simulink model "myo_sfun_one_myo_imu_emg"  (R2019a)
settings: Solver=ode1  StartTime=0.0  StopTime=inf  FixedStep=0.005  RelTol=1e-3  EnableMultiTasking=on
libraries: neural x1018, myo_lib x2, sldrtlib x1, dspnetwork x1
(part 4 of 12)

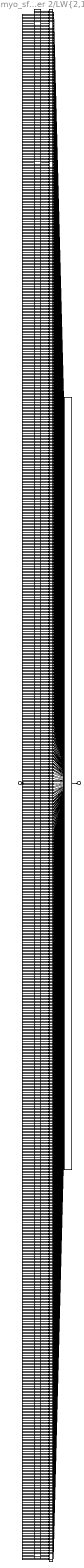
== system myo_sfun_one_myo_imu_emg/Pattern Recognition Neural Network/Layer 2/LW{2,1} ==
  "ad{2,1}" : Inport  PortDimensions=8
      mask Display: e = 0.06;c1 = [120 230 180]/255;c2 = ([120 230 180]+0)/(256+128);c3 = ([120 230 180]+128)/(256+128);patch([0 1 1 0],[0 0 1 1],c1);patch([0 1 1 1-e 1-e 0+e],[0 0 1 1-e 0+e 0+e],c2);patch([0 0 1 1-e 0+e 0+e],[0 1 1 1-e 1-e 0+e],c3);plot([0 1 1 0 0],[0 0 1 1 0]);
  "IW{2,1}(1,:)'" : Constant  Value=[-0.691660917205364711435322533361613750457763671875;-1.7584420611645865673011712715378962457180023193359375;-1.7122805471842796887216309187351725995540618896484375;0.1557580120848369997776927675658953376114368438720703125;-1.4322595499423294018725982823525555431842803955078125;-1.0116917192643277711994187484378926455974578857421875;0.60338568391011870861717625302844680845737457275390625;-1.10261377542594374290274572558701038360595703125]
      mask Display: e = 0.06;c1 = [120 150 230]/255;c2 = ([120 150 230]+0)/383;c3 = ([120 150 230]+128)/383;patch([0 1 1 0],[0 0 1 1],c1);patch([0 1 1 1-e 1-e 0+e],[0 0 1 1-e 0+e 0+e],c2);patch([0 0 1 1-e 0+e 0+e],[0 1 1 1-e 1-e 0+e],c3);plot([0 1 1 0 0],[0 0 1 1 0]);disp('weights');
  "IW{2,1}(10,:)'" : Constant  Value=[0.29748051894865035205128833695198409259319305419921875;-1.4335889907109626850711947554373182356357574462890625;0.162112670099137046175741261322400532662868499755859375;-1.5012829071378430700889339277637191116809844970703125;2.075601849797474418579668054007925093173980712890625;1.3052358877568857042916761201922781765460968017578125;0.2314436321550090436272029137398931197822093963623046875;-0.75565891962408227033876073619467206299304962158203125]
      mask Display: e = 0.06;c1 = [120 150 230]/255;c2 = ([120 150 230]+0)/383;c3 = ([120 150 230]+128)/383;patch([0 1 1 0],[0 0 1 1],c1);patch([0 1 1 1-e 1-e 0+e],[0 0 1 1-e 0+e 0+e],c2);patch([0 0 1 1-e 0+e 0+e],[0 1 1 1-e 1-e 0+e],c3);plot([0 1 1 0 0],[0 0 1 1 0]);disp('weights');
  "IW{2,1}(100,:)'" : Constant  Value=[-0.1965433836533932165924198898210306651890277862548828125;-0.694918414161374897730638622306287288665771484375;0.66443928778979233218393574134097434580326080322265625;0.4810398818895180728105742673506028950214385986328125;-0.77850581457315548572495345069910399615764617919921875;-1.77609819693787951422336846007965505123138427734375;1.4679904515706148071529923981870524585247039794921875;-1.944332630962620545034269525785930454730987548828125]
      mask Display: e = 0.06;c1 = [120 150 230]/255;c2 = ([120 150 230]+0)/383;c3 = ([120 150 230]+128)/383;patch([0 1 1 0],[0 0 1 1],c1);patch([0 1 1 1-e 1-e 0+e],[0 0 1 1-e 0+e 0+e],c2);patch([0 0 1 1-e 0+e 0+e],[0 1 1 1-e 1-e 0+e],c3);plot([0 1 1 0 0],[0 0 1 1 0]);disp('weights');
  "IW{2,1}(1000,:)'" : Constant  Value=[-0.75896391948230645940753902323194779455661773681640625;1.8795374511604172607093232727493159472942352294921875;1.5450884416724310899127203811076469719409942626953125;0.98730253999568906575490245813853107392787933349609375;0.54160434848503913318751301630982197821140289306640625;-1.3842186077384701636816544123576022684574127197265625;-1.0252246817422523417207003149087540805339813232421875;-0.61302757920082961984320490955724380910396575927734375]
      mask Display: e = 0.06;c1 = [120 150 230]/255;c2 = ([120 150 230]+0)/383;c3 = ([120 150 230]+128)/383;patch([0 1 1 0],[0 0 1 1],c1);patch([0 1 1 1-e 1-e 0+e],[0 0 1 1-e 0+e 0+e],c2);patch([0 0 1 1-e 0+e 0+e],[0 1 1 1-e 1-e 0+e],c3);plot([0 1 1 0 0],[0 0 1 1 0]);disp('weights');
  "IW{2,1}(101,:)'" : Constant  Value=[-0.7346292753484846560496634992887265980243682861328125;1.6733957934261258770902713877148926258087158203125;-0.93987189965385997680868968018330633640289306640625;-2.098880370538726225504433386959135532379150390625;0.41553672602720481688010067955474369227886199951171875;0.483898246991799119154364916539634577929973602294921875;-1.4358615101881204711986583788529969751834869384765625;-0.5692919905849540551656673414981923997402191162109375]
      mask Display: e = 0.06;c1 = [120 150 230]/255;c2 = ([120 150 230]+0)/383;c3 = ([120 150 230]+128)/383;patch([0 1 1 0],[0 0 1 1],c1);patch([0 1 1 1-e 1-e 0+e],[0 0 1 1-e 0+e 0+e],c2);patch([0 0 1 1-e 0+e 0+e],[0 1 1 1-e 1-e 0+e],c3);plot([0 1 1 0 0],[0 0 1 1 0]);disp('weights');
  "IW{2,1}(102,:)'" : Constant  Value=[-0.752794916939543146128244188730604946613311767578125;1.166938084302759026655849083908833563327789306640625;2.171459819669392832253151937038637697696685791015625;0.55570154129463655845455605231109075248241424560546875;1.7372623920478691417201844160445034503936767578125;-0.1828342599738930207564635566086508333683013916015625;0.617021132023727769677634569234214723110198974609375;-0.798583301335380912888695092988200485706329345703125]
      mask Display: e = 0.06;c1 = [120 150 230]/255;c2 = ([120 150 230]+0)/383;c3 = ([120 150 230]+128)/383;patch([0 1 1 0],[0 0 1 1],c1);patch([0 1 1 1-e 1-e 0+e],[0 0 1 1-e 0+e 0+e],c2);patch([0 0 1 1-e 0+e 0+e],[0 1 1 1-e 1-e 0+e],c3);plot([0 1 1 0 0],[0 0 1 1 0]);disp('weights');
  "IW{2,1}(103,:)'" : Constant  Value=[-1.1068634406180850593415243565686978399753570556640625;-0.68329593258649257148107380999135784804821014404296875;0.9236877373804779356447625104920007288455963134765625;-0.79483289464276729585634484465117566287517547607421875;-1.36336981772248311273187937331385910511016845703125;-1.6712995505896552916880182237946428358554840087890625;-1.63520965259610573383497467148117721080780029296875;0.7975112275656390803391104782349430024623870849609375]
      mask Display: e = 0.06;c1 = [120 150 230]/255;c2 = ([120 150 230]+0)/383;c3 = ([120 150 230]+128)/383;patch([0 1 1 0],[0 0 1 1],c1);patch([0 1 1 1-e 1-e 0+e],[0 0 1 1-e 0+e 0+e],c2);patch([0 0 1 1-e 0+e 0+e],[0 1 1 1-e 1-e 0+e],c3);plot([0 1 1 0 0],[0 0 1 1 0]);disp('weights');
  "IW{2,1}(104,:)'" : Constant  Value=[-1.2039908850799425632516204132116399705410003662109375;-1.722550343662703209446362961898557841777801513671875;-0.733634489926349164790053691831417381763458251953125;1.482941468037298538007462411769665777683258056640625;0.0976439227042145974078124481820850633084774017333984375;-1.577352115355438844090940619935281574726104736328125;0.4027722868890502017080734731280244886875152587890625;1.4632670973491415100653512126882560551166534423828125]
      mask Display: e = 0.06;c1 = [120 150 230]/255;c2 = ([120 150 230]+0)/383;c3 = ([120 150 230]+128)/383;patch([0 1 1 0],[0 0 1 1],c1);patch([0 1 1 1-e 1-e 0+e],[0 0 1 1-e 0+e 0+e],c2);patch([0 0 1 1-e 0+e 0+e],[0 1 1 1-e 1-e 0+e],c3);plot([0 1 1 0 0],[0 0 1 1 0]);disp('weights');
  "IW{2,1}(105,:)'" : Constant  Value=[-0.82970148356722717153388657607138156890869140625;1.476196773208704460245144218788482248783111572265625;-0.84817603974084032625313511744025163352489471435546875;-1.357590893906548412672918857424519956111907958984375;1.9196514396686323866703105522901751101016998291015625;0.51783204664954884943739443770027719438076019287109375;0.166333228616280137668326233324478380382061004638671875;1.2661311610600314292440771168912760913372039794921875]
      mask Display: e = 0.06;c1 = [120 150 230]/255;c2 = ([120 150 230]+0)/383;c3 = ([120 150 230]+128)/383;patch([0 1 1 0],[0 0 1 1],c1);patch([0 1 1 1-e 1-e 0+e],[0 0 1 1-e 0+e 0+e],c2);patch([0 0 1 1-e 0+e 0+e],[0 1 1 1-e 1-e 0+e],c3);plot([0 1 1 0 0],[0 0 1 1 0]);disp('weights');
  "IW{2,1}(106,:)'" : Constant  Value=[-2.049359601734397795524955654400400817394256591796875;-1.665285450772149733467131227371282875537872314453125;0.87993744188790279370238067713216878473758697509765625;-1.5679190268193672341823230453883297741413116455078125;0.36094306234647299813644849564298056066036224365234375;-0.0369441453771053307519878217135556042194366455078125;0.0216282674490956665358520893960303510539233684539794921875;-0.99199514984426906405445834025158546864986419677734375]
      mask Display: e = 0.06;c1 = [120 150 230]/255;c2 = ([120 150 230]+0)/383;c3 = ([120 150 230]+128)/383;patch([0 1 1 0],[0 0 1 1],c1);patch([0 1 1 1-e 1-e 0+e],[0 0 1 1-e 0+e 0+e],c2);patch([0 0 1 1-e 0+e 0+e],[0 1 1 1-e 1-e 0+e],c3);plot([0 1 1 0 0],[0 0 1 1 0]);disp('weights');
  "IW{2,1}(107,:)'" : Constant  Value=[1.526235863593053299069879358285106718540191650390625;-1.2098465596567213875545121481991373002529144287109375;-0.3327773356104037905112136286334134638309478759765625;1.6991612055741971420985692020622082054615020751953125;-1.4350855371585951036905726141412742435932159423828125;0.09974716737212674377843768525053746998310089111328125;-1.0362891110155614260435186224640347063541412353515625;1.13218572804818240484792113420553505420684814453125]
      mask Display: e = 0.06;c1 = [120 150 230]/255;c2 = ([120 150 230]+0)/383;c3 = ([120 150 230]+128)/383;patch([0 1 1 0],[0 0 1 1],c1);patch([0 1 1 1-e 1-e 0+e],[0 0 1 1-e 0+e 0+e],c2);patch([0 0 1 1-e 0+e 0+e],[0 1 1 1-e 1-e 0+e],c3);plot([0 1 1 0 0],[0 0 1 1 0]);disp('weights');
  "IW{2,1}(108,:)'" : Constant  Value=[-0.8124994162632557248571174568496644496917724609375;-1.5665539983796381573455391844618134200572967529296875;-0.187224386217166360868446872700587846338748931884765625;1.0861775880444961561721584075712598860263824462890625;1.351917275444545651907901628874242305755615234375;-0.83378037725782350175762758226483128964900970458984375;-1.385421527250217277327237752615474164485931396484375;1.5546422525807359615868108448921702802181243896484375]
      mask Display: e = 0.06;c1 = [120 150 230]/255;c2 = ([120 150 230]+0)/383;c3 = ([120 150 230]+128)/383;patch([0 1 1 0],[0 0 1 1],c1);patch([0 1 1 1-e 1-e 0+e],[0 0 1 1-e 0+e 0+e],c2);patch([0 0 1 1-e 0+e 0+e],[0 1 1 1-e 1-e 0+e],c3);plot([0 1 1 0 0],[0 0 1 1 0]);disp('weights');
  "IW{2,1}(109,:)'" : Constant  Value=[0.19012578102685784298131466130143962800502777099609375;1.44821196542192875966748033533804118633270263671875;-0.669229510490122248000943727674894034862518310546875;1.3059840050621274176734232241869904100894927978515625;-0.8163339678271857025038116262294352054595947265625;-1.4775762628706907708675544199650175869464874267578125;0.87987224253331641765640824814909137785434722900390625;1.6788826743721418921495569520629942417144775390625]
      mask Display: e = 0.06;c1 = [120 150 230]/255;c2 = ([120 150 230]+0)/383;c3 = ([120 150 230]+128)/383;patch([0 1 1 0],[0 0 1 1],c1);patch([0 1 1 1-e 1-e 0+e],[0 0 1 1-e 0+e 0+e],c2);patch([0 0 1 1-e 0+e 0+e],[0 1 1 1-e 1-e 0+e],c3);plot([0 1 1 0 0],[0 0 1 1 0]);disp('weights');
  "IW{2,1}(11,:)'" : Constant  Value=[2.091364144074137954021352925337851047515869140625;1.19190169735374329462729292572475969791412353515625;0.438539695265063256268689428907237015664577484130859375;1.427779135746976901799598635989241302013397216796875;-1.1734334596731803568303575957543216645717620849609375;-0.75612406354167938093979728364502079784870147705078125;-0.85559840138312071022852478563436307013034820556640625;0.6340354257080207389662973582744598388671875]
      mask Display: e = 0.06;c1 = [120 150 230]/255;c2 = ([120 150 230]+0)/383;c3 = ([120 150 230]+128)/383;patch([0 1 1 0],[0 0 1 1],c1);patch([0 1 1 1-e 1-e 0+e],[0 0 1 1-e 0+e 0+e],c2);patch([0 0 1 1-e 0+e 0+e],[0 1 1 1-e 1-e 0+e],c3);plot([0 1 1 0 0],[0 0 1 1 0]);disp('weights');
  "IW{2,1}(110,:)'" : Constant  Value=[1.12310065411607507002145212027244269847869873046875;0.65381754150688775606425906516960822045803070068359375;0.483190932248633464585196861662552691996097564697265625;1.5216055898993252615269966554478742182254791259765625;-1.618210254067223186069668372510932385921478271484375;-0.8486399726322251257926154721644707024097442626953125;0.424500550557350420088909004334709607064723968505859375;1.760175767722318429520100835361517965793609619140625]
      mask Display: e = 0.06;c1 = [120 150 230]/255;c2 = ([120 150 230]+0)/383;c3 = ([120 150 230]+128)/383;patch([0 1 1 0],[0 0 1 1],c1);patch([0 1 1 1-e 1-e 0+e],[0 0 1 1-e 0+e 0+e],c2);patch([0 0 1 1-e 0+e 0+e],[0 1 1 1-e 1-e 0+e],c3);plot([0 1 1 0 0],[0 0 1 1 0]);disp('weights');
  "IW{2,1}(111,:)'" : Constant  Value=[-1.45835723777261261346893661539070308208465576171875;0.460958016356734834317876448039896786212921142578125;0.82960262943399343260608702621539123356342315673828125;1.764946563170818993881994174444116652011871337890625;1.867300072530361010336719118640758097171783447265625;0.4866543505420615201018108564312569797039031982421875;0.47638255663761619462803764690761454403400421142578125;0.967658595669160792596130704623647034168243408203125]
      mask Display: e = 0.06;c1 = [120 150 230]/255;c2 = ([120 150 230]+0)/383;c3 = ([120 150 230]+128)/383;patch([0 1 1 0],[0 0 1 1],c1);patch([0 1 1 1-e 1-e 0+e],[0 0 1 1-e 0+e 0+e],c2);patch([0 0 1 1-e 0+e 0+e],[0 1 1 1-e 1-e 0+e],c3);plot([0 1 1 0 0],[0 0 1 1 0]);disp('weights');
  "IW{2,1}(112,:)'" : Constant  Value=[0.90630292675991774853372362485970370471477508544921875;-0.7483178408217094901289101471775211393833160400390625;-1.4719554269169139448791838731267489492893218994140625;-1.3185905102969688318381713543203659355640411376953125;1.11248064428886461740830782218836247920989990234375;-1.902432566793907486868420164682902395725250244140625;0.80968802704409836845655945580801926553249359130859375;0.471445922634182945643033235683105885982513427734375]
      mask Display: e = 0.06;c1 = [120 150 230]/255;c2 = ([120 150 230]+0)/383;c3 = ([120 150 230]+128)/383;patch([0 1 1 0],[0 0 1 1],c1);patch([0 1 1 1-e 1-e 0+e],[0 0 1 1-e 0+e 0+e],c2);patch([0 0 1 1-e 0+e 0+e],[0 1 1 1-e 1-e 0+e],c3);plot([0 1 1 0 0],[0 0 1 1 0]);disp('weights');
  "IW{2,1}(113,:)'" : Constant  Value=[-2.1700138842824419072030650568194687366485595703125;-1.2265632677169240327685884039965458214282989501953125;0.31278242318674431832192794900038279592990875244140625;-1.17937237170043918155215578735806047916412353515625;0.495421493364235576706278152414597570896148681640625;1.579508580603393941288459245697595179080963134765625;-0.435311629212086825813088353243074379861354827880859375;0.6223682610868095377298914172570221126079559326171875]
      mask Display: e = 0.06;c1 = [120 150 230]/255;c2 = ([120 150 230]+0)/383;c3 = ([120 150 230]+128)/383;patch([0 1 1 0],[0 0 1 1],c1);patch([0 1 1 1-e 1-e 0+e],[0 0 1 1-e 0+e 0+e],c2);patch([0 0 1 1-e 0+e 0+e],[0 1 1 1-e 1-e 0+e],c3);plot([0 1 1 0 0],[0 0 1 1 0]);disp('weights');
  "IW{2,1}(114,:)'" : Constant  Value=[-0.95960652512177302408957757506868802011013031005859375;-1.171099316170392423686053007259033620357513427734375;1.2005938613692059835358350028400309383869171142578125;-1.0271322442187591494899834287934936583042144775390625;0.275734884241691513562244608692708425223827362060546875;-2.273917403532263126209045367431826889514923095703125;0.60594431945872850864276415450149215757846832275390625;0.788812091891621047778926367755047976970672607421875]
      mask Display: e = 0.06;c1 = [120 150 230]/255;c2 = ([120 150 230]+0)/383;c3 = ([120 150 230]+128)/383;patch([0 1 1 0],[0 0 1 1],c1);patch([0 1 1 1-e 1-e 0+e],[0 0 1 1-e 0+e 0+e],c2);patch([0 0 1 1-e 0+e 0+e],[0 1 1 1-e 1-e 0+e],c3);plot([0 1 1 0 0],[0 0 1 1 0]);disp('weights');
  "IW{2,1}(115,:)'" : Constant  Value=[1.259842960302490322277435552678070962429046630859375;1.7763440982486831121178738612798042595386505126953125;1.7368956039236851385254567503579892218112945556640625;0.489479457804314399549383551857317797839641571044921875;-0.69836997846389603505912191394600085914134979248046875;-0.69450858609234611407146076089702546596527099609375;-1.584018966753015345005906056030653417110443115234375;-0.143556776088628101906152778610703535377979278564453125]
      mask Display: e = 0.06;c1 = [120 150 230]/255;c2 = ([120 150 230]+0)/383;c3 = ([120 150 230]+128)/383;patch([0 1 1 0],[0 0 1 1],c1);patch([0 1 1 1-e 1-e 0+e],[0 0 1 1-e 0+e 0+e],c2);patch([0 0 1 1-e 0+e 0+e],[0 1 1 1-e 1-e 0+e],c3);plot([0 1 1 0 0],[0 0 1 1 0]);disp('weights');
  "IW{2,1}(116,:)'" : Constant  Value=[1.1305890114884669106487535827909596264362335205078125;-0.2309211402775909471873916345430188812315464019775390625;1.4467085200288185564687637452152557671070098876953125;1.683074804270280555584804460522718727588653564453125;-1.10822346900712087602869360125623643398284912109375;1.3197346249344026336558499679085798561573028564453125;0.19679073836889859894228038683650083839893341064453125;-1.310618823194344084726026267162524163722991943359375]
      mask Display: e = 0.06;c1 = [120 150 230]/255;c2 = ([120 150 230]+0)/383;c3 = ([120 150 230]+128)/383;patch([0 1 1 0],[0 0 1 1],c1);patch([0 1 1 1-e 1-e 0+e],[0 0 1 1-e 0+e 0+e],c2);patch([0 0 1 1-e 0+e 0+e],[0 1 1 1-e 1-e 0+e],c3);plot([0 1 1 0 0],[0 0 1 1 0]);disp('weights');
  "IW{2,1}(117,:)'" : Constant  Value=[-1.2965092749014439643673313184990547597408294677734375;-0.40909004021247497018265448787133209407329559326171875;0.232380826221318004254356992532848380506038665771484375;-1.4938038430410289780780885848798789083957672119140625;-1.4111858515245507827984283721889369189739227294921875;-1.3798668297073295452292995832976885139942169189453125;-0.5736035650808333219430323879350908100605010986328125;1.545401209062778224989642694708891212940216064453125]
      mask Display: e = 0.06;c1 = [120 150 230]/255;c2 = ([120 150 230]+0)/383;c3 = ([120 150 230]+128)/383;patch([0 1 1 0],[0 0 1 1],c1);patch([0 1 1 1-e 1-e 0+e],[0 0 1 1-e 0+e 0+e],c2);patch([0 0 1 1-e 0+e 0+e],[0 1 1 1-e 1-e 0+e],c3);plot([0 1 1 0 0],[0 0 1 1 0]);disp('weights');
  "IW{2,1}(118,:)'" : Constant  Value=[-0.431220772164270016446607769466936588287353515625;1.4980663049915936557709983389941044151782989501953125;-0.032124284553384778451157188783327001146972179412841796875;-0.99178065612847543519592363736592233180999755859375;-0.90983063362129545925682805318501777946949005126953125;-0.94491687952873892886174189698067493736743927001953125;0.2190608048581546840605227544074296019971370697021484375;2.4177856342907144693299414939247071743011474609375]
      mask Display: e = 0.06;c1 = [120 150 230]/255;c2 = ([120 150 230]+0)/383;c3 = ([120 150 230]+128)/383;patch([0 1 1 0],[0 0 1 1],c1);patch([0 1 1 1-e 1-e 0+e],[0 0 1 1-e 0+e 0+e],c2);patch([0 0 1 1-e 0+e 0+e],[0 1 1 1-e 1-e 0+e],c3);plot([0 1 1 0 0],[0 0 1 1 0]);disp('weights');
  "IW{2,1}(119,:)'" : Constant  Value=[2.032289941457469328867091462598182260990142822265625;1.2300087485055588576443597048637457191944122314453125;1.1312373102641062327933241249411366879940032958984375;-1.366286246477192545256684752530418336391448974609375;-0.392858662961971472071809330373071134090423583984375;1.3600255209509413134583155624568462371826171875;-0.4417275309143331440964175271801650524139404296875;-0.64492461423233715667180376840406097471714019775390625]
      mask Display: e = 0.06;c1 = [120 150 230]/255;c2 = ([120 150 230]+0)/383;c3 = ([120 150 230]+128)/383;patch([0 1 1 0],[0 0 1 1],c1);patch([0 1 1 1-e 1-e 0+e],[0 0 1 1-e 0+e 0+e],c2);patch([0 0 1 1-e 0+e 0+e],[0 1 1 1-e 1-e 0+e],c3);plot([0 1 1 0 0],[0 0 1 1 0]);disp('weights');
  "IW{2,1}(12,:)'" : Constant  Value=[0.91486769312648663632359102848567999899387359619140625;0.56602701691960033425488063585362397134304046630859375;-1.25438509677780274387259851209819316864013671875;-0.63813074054059371054137272949446924030780792236328125;-1.363451099083925033284003802691586315631866455078125;-0.0252649558450613286042507610318352817557752132415771484375;-2.32042882861984889331097292597405612468719482421875;0.80044852883130257481525404728017747402191162109375]
      mask Display: e = 0.06;c1 = [120 150 230]/255;c2 = ([120 150 230]+0)/383;c3 = ([120 150 230]+128)/383;patch([0 1 1 0],[0 0 1 1],c1);patch([0 1 1 1-e 1-e 0+e],[0 0 1 1-e 0+e 0+e],c2);patch([0 0 1 1-e 0+e 0+e],[0 1 1 1-e 1-e 0+e],c3);plot([0 1 1 0 0],[0 0 1 1 0]);disp('weights');
  "IW{2,1}(120,:)'" : Constant  Value=[0.42250540399770775135124267762876115739345550537109375;1.7440741240887638330292475075111724436283111572265625;1.45134468863258181414721548208035528659820556640625;-0.94540168936672552835176475127809680998325347900390625;1.349986197984198721400161957717500627040863037109375;-0.65996498605669351444902304137940518558025360107421875;-1.73587667519844845998022719868458807468414306640625;0.59414197129898915772372447463567368686199188232421875]
      mask Display: e = 0.06;c1 = [120 150 230]/255;c2 = ([120 150 230]+0)/383;c3 = ([120 150 230]+128)/383;patch([0 1 1 0],[0 0 1 1],c1);patch([0 1 1 1-e 1-e 0+e],[0 0 1 1-e 0+e 0+e],c2);patch([0 0 1 1-e 0+e 0+e],[0 1 1 1-e 1-e 0+e],c3);plot([0 1 1 0 0],[0 0 1 1 0]);disp('weights');
  "IW{2,1}(121,:)'" : Constant  Value=[0.2953824440974088805234032406588084995746612548828125;0.19947891835721265341163643824984319508075714111328125;-1.7008412375581887232556255185045301914215087890625;-0.70194035735294824096541788094327785074710845947265625;2.00078921034554024771523472736589610576629638671875;-0.171731474879736278893460621475242078304290771484375;0.57037505385167686089431526852422393858432769775390625;1.6685824846776340368847968420595861971378326416015625]
      mask Display: e = 0.06;c1 = [120 150 230]/255;c2 = ([120 150 230]+0)/383;c3 = ([120 150 230]+128)/383;patch([0 1 1 0],[0 0 1 1],c1);patch([0 1 1 1-e 1-e 0+e],[0 0 1 1-e 0+e 0+e],c2);patch([0 0 1 1-e 0+e 0+e],[0 1 1 1-e 1-e 0+e],c3);plot([0 1 1 0 0],[0 0 1 1 0]);disp('weights');
  "IW{2,1}(122,:)'" : Constant  Value=[2.389346377458451797792804427444934844970703125;1.8579702943205924636771442237659357488155364990234375;-1.24041157938239177127570656011812388896942138671875;-0.312204907514915308563985263390350155532360076904296875;0.47345305603977294595097191631793975830078125;0.08085799640160480639128337543297675438225269317626953125;0.425169260567675622031202919970382936298847198486328125;-0.58418175654939208385485471808351576328277587890625]
      mask Display: e = 0.06;c1 = [120 150 230]/255;c2 = ([120 150 230]+0)/383;c3 = ([120 150 230]+128)/383;patch([0 1 1 0],[0 0 1 1],c1);patch([0 1 1 1-e 1-e 0+e],[0 0 1 1-e 0+e 0+e],c2);patch([0 0 1 1-e 0+e 0+e],[0 1 1 1-e 1-e 0+e],c3);plot([0 1 1 0 0],[0 0 1 1 0]);disp('weights');
  "IW{2,1}(123,:)'" : Constant  Value=[0.87447765532420562717419443288235925137996673583984375;-1.404484008896221158835260212072171270847320556640625;0.066383199277035453977902079714112915098667144775390625;-2.14177965994965813223416262189857661724090576171875;-0.35409024524090426666589337401092052459716796875;-0.8321991451194150624104395319591276347637176513671875;-0.1303406369226948469108862127541215158998966217041015625;-1.6968377321111436373257674858905375003814697265625]
      mask Display: e = 0.06;c1 = [120 150 230]/255;c2 = ([120 150 230]+0)/383;c3 = ([120 150 230]+128)/383;patch([0 1 1 0],[0 0 1 1],c1);patch([0 1 1 1-e 1-e 0+e],[0 0 1 1-e 0+e 0+e],c2);patch([0 0 1 1-e 0+e 0+e],[0 1 1 1-e 1-e 0+e],c3);plot([0 1 1 0 0],[0 0 1 1 0]);disp('weights');
  "IW{2,1}(124,:)'" : Constant  Value=[-1.20468773335336098995185238891281187534332275390625;-0.86840097966744733692934232749394141137599945068359375;0.5244983963447131802837475333944894373416900634765625;-1.4107774861939119670495301761548034846782684326171875;1.4946368323390231136471584250102750957012176513671875;-1.358016823143335383150542838848195970058441162109375;-0.63820615731996588326779829003498889505863189697265625;-1.41402043973897217910007384489290416240692138671875]
      mask Display: e = 0.06;c1 = [120 150 230]/255;c2 = ([120 150 230]+0)/383;c3 = ([120 150 230]+128)/383;patch([0 1 1 0],[0 0 1 1],c1);patch([0 1 1 1-e 1-e 0+e],[0 0 1 1-e 0+e 0+e],c2);patch([0 0 1 1-e 0+e 0+e],[0 1 1 1-e 1-e 0+e],c3);plot([0 1 1 0 0],[0 0 1 1 0]);disp('weights');
  "IW{2,1}(125,:)'" : Constant  Value=[-0.506779246737117272658679212327115237712860107421875;0.08469404380268320819968863588655949570238590240478515625;0.96661146073616155405261451960541307926177978515625;2.21984576565986291285526021965779364109039306640625;-0.325247928172124389778474551349063403904438018798828125;-2.141187307560778574355708769871853291988372802734375;0.14891670820092250959731927650864236056804656982421875;0.63327011999696491972855483254534192383289337158203125]
      mask Display: e = 0.06;c1 = [120 150 230]/255;c2 = ([120 150 230]+0)/383;c3 = ([120 150 230]+128)/383;patch([0 1 1 0],[0 0 1 1],c1);patch([0 1 1 1-e 1-e 0+e],[0 0 1 1-e 0+e 0+e],c2);patch([0 0 1 1-e 0+e 0+e],[0 1 1 1-e 1-e 0+e],c3);plot([0 1 1 0 0],[0 0 1 1 0]);disp('weights');
  "IW{2,1}(126,:)'" : Constant  Value=[1.954875514761962307375142700038850307464599609375;0.7484979057490068754532330785878002643585205078125;0.1966880304213210750585716368732391856610774993896484375;-0.23710090993159138594847945569199509918689727783203125;1.134606059769200481213147213566116988658905029296875;2.2163351976999177139759922283701598644256591796875;0.361245693778591447919978918434935621917247772216796875;0.29868377131698398141423922425019554793834686279296875]
      mask Display: e = 0.06;c1 = [120 150 230]/255;c2 = ([120 150 230]+0)/383;c3 = ([120 150 230]+128)/383;patch([0 1 1 0],[0 0 1 1],c1);patch([0 1 1 1-e 1-e 0+e],[0 0 1 1-e 0+e 0+e],c2);patch([0 0 1 1-e 0+e 0+e],[0 1 1 1-e 1-e 0+e],c3);plot([0 1 1 0 0],[0 0 1 1 0]);disp('weights');
  "IW{2,1}(127,:)'" : Constant  Value=[0.7694262528917914512049947006744332611560821533203125;0.858673114136447868105506131541915237903594970703125;-1.9591912322259281697967026047990657389163970947265625;0.7765373081231425889114916571998037397861480712890625;-2.12514482442326624322959105484187602996826171875;-0.51247220026288908822920120655908249318599700927734375;0.66660374982875791882719340719631873071193695068359375;0.2215181162421060445666398663888685405254364013671875]
      mask Display: e = 0.06;c1 = [120 150 230]/255;c2 = ([120 150 230]+0)/383;c3 = ([120 150 230]+128)/383;patch([0 1 1 0],[0 0 1 1],c1);patch([0 1 1 1-e 1-e 0+e],[0 0 1 1-e 0+e 0+e],c2);patch([0 0 1 1-e 0+e 0+e],[0 1 1 1-e 1-e 0+e],c3);plot([0 1 1 0 0],[0 0 1 1 0]);disp('weights');
  "IW{2,1}(128,:)'" : Constant  Value=[-0.4645036239519015897059261988033540546894073486328125;0.0578363955944476149095834216495859436690807342529296875;0.79269376078468878343841197420260868966579437255859375;-0.8815416918189125095040026280912570655345916748046875;0.1192744047821424902000586598660447634756565093994140625;2.060366205871878353406145834014751017093658447265625;-1.99426682885684503077072804444469511508941650390625;-1.1547872117878557052250698689022101461887359619140625]
      mask Display: e = 0.06;c1 = [120 150 230]/255;c2 = ([120 150 230]+0)/383;c3 = ([120 150 230]+128)/383;patch([0 1 1 0],[0 0 1 1],c1);patch([0 1 1 1-e 1-e 0+e],[0 0 1 1-e 0+e 0+e],c2);patch([0 0 1 1-e 0+e 0+e],[0 1 1 1-e 1-e 0+e],c3);plot([0 1 1 0 0],[0 0 1 1 0]);disp('weights');
  "IW{2,1}(129,:)'" : Constant  Value=[-1.7954776257203086675673375793849118053913116455078125;-0.77067172361155000803734083092422224581241607666015625;-1.5025825472358846912612762025673873722553253173828125;-1.474556982392986714813787330058403313159942626953125;0.12129332666747798252782075678624096326529979705810546875;-0.462321049146925344697223181356093846261501312255859375;1.33241983510785733102466110722161829471588134765625;-0.472279832509858110700662336967070586979389190673828125]
      mask Display: e = 0.06;c1 = [120 150 230]/255;c2 = ([120 150 230]+0)/383;c3 = ([120 150 230]+128)/383;patch([0 1 1 0],[0 0 1 1],c1);patch([0 1 1 1-e 1-e 0+e],[0 0 1 1-e 0+e 0+e],c2);patch([0 0 1 1-e 0+e 0+e],[0 1 1 1-e 1-e 0+e],c3);plot([0 1 1 0 0],[0 0 1 1 0]);disp('weights');
  "IW{2,1}(13,:)'" : Constant  Value=[1.4722183686413501391143654473125934600830078125;-1.4533406460287687789190158582641743123531341552734375;-1.6756603659175632881073170210584066808223724365234375;0.1239486161395557950459789253727649338543415069580078125;1.065594255147046975906732768635265529155731201171875;-0.455146428364095967378233353883842937648296356201171875;0.2143238030204172861470368616210180334746837615966796875;-1.5942987059197886168249169713817536830902099609375]
      mask Display: e = 0.06;c1 = [120 150 230]/255;c2 = ([120 150 230]+0)/383;c3 = ([120 150 230]+128)/383;patch([0 1 1 0],[0 0 1 1],c1);patch([0 1 1 1-e 1-e 0+e],[0 0 1 1-e 0+e 0+e],c2);patch([0 0 1 1-e 0+e 0+e],[0 1 1 1-e 1-e 0+e],c3);plot([0 1 1 0 0],[0 0 1 1 0]);disp('weights');
  "IW{2,1}(130,:)'" : Constant  Value=[-0.55363441841454597014404725996428169310092926025390625;0.95680857713087352767189486257848329842090606689453125;-1.255947108543568280225599664845503866672515869140625;2.021771324134128189342618497903458774089813232421875;-0.061796225740531542103273210386760183610022068023681640625;2.0317171954915966836097140912897884845733642578125;0.020301648902267176166613893428802839480340480804443359375;0.07304264326480751357006937496407772414386272430419921875]
      mask Display: e = 0.06;c1 = [120 150 230]/255;c2 = ([120 150 230]+0)/383;c3 = ([120 150 230]+128)/383;patch([0 1 1 0],[0 0 1 1],c1);patch([0 1 1 1-e 1-e 0+e],[0 0 1 1-e 0+e 0+e],c2);patch([0 0 1 1-e 0+e 0+e],[0 1 1 1-e 1-e 0+e],c3);plot([0 1 1 0 0],[0 0 1 1 0]);disp('weights');
  "IW{2,1}(131,:)'" : Constant  Value=[-2.180474603917020193222242596675641834735870361328125;0.72645735914720344084116732119582593441009521484375;1.018870908321010571029319180524908006191253662109375;1.383323172901160358350125534343533217906951904296875;0.4625022964292087035431677577435038983821868896484375;0.64331250774203974085452273357077501714229583740234375;1.0715339161900170328323156354599632322788238525390625;-1.0219064363191299182886950802640058100223541259765625]
      mask Display: e = 0.06;c1 = [120 150 230]/255;c2 = ([120 150 230]+0)/383;c3 = ([120 150 230]+128)/383;patch([0 1 1 0],[0 0 1 1],c1);patch([0 1 1 1-e 1-e 0+e],[0 0 1 1-e 0+e 0+e],c2);patch([0 0 1 1-e 0+e 0+e],[0 1 1 1-e 1-e 0+e],c3);plot([0 1 1 0 0],[0 0 1 1 0]);disp('weights');
  "IW{2,1}(132,:)'" : Constant  Value=[0.75489337030717684751124352260376326739788055419921875;-0.782732462432700781818084578844718635082244873046875;0.5931203619410660987654182463302277028560638427734375;0.9184312361182238593215743094333447515964508056640625;-0.42386247367815510500577147467993199825286865234375;1.56965304535986671652381119201891124248504638671875;1.6982589389750326613892639215919189155101776123046875;1.750190304231196147810578622738830745220184326171875]
      mask Display: e = 0.06;c1 = [120 150 230]/255;c2 = ([120 150 230]+0)/383;c3 = ([120 150 230]+128)/383;patch([0 1 1 0],[0 0 1 1],c1);patch([0 1 1 1-e 1-e 0+e],[0 0 1 1-e 0+e 0+e],c2);patch([0 0 1 1-e 0+e 0+e],[0 1 1 1-e 1-e 0+e],c3);plot([0 1 1 0 0],[0 0 1 1 0]);disp('weights');
  "IW{2,1}(133,:)'" : Constant  Value=[0.7123465712444403408198922988958656787872314453125;2.361424615797688364438045027782209217548370361328125;1.903559317488005664387173965224064886569976806640625;-0.11361441222337249901119804462723550386726856231689453125;0.68170139583434796737293481783126480877399444580078125;0.1784087551198940968522066441437345929443836212158203125;-0.468471511711015142775949016140657477080821990966796875;-0.807410088487492405562306885258294641971588134765625]
      mask Display: e = 0.06;c1 = [120 150 230]/255;c2 = ([120 150 230]+0)/383;c3 = ([120 150 230]+128)/383;patch([0 1 1 0],[0 0 1 1],c1);patch([0 1 1 1-e 1-e 0+e],[0 0 1 1-e 0+e 0+e],c2);patch([0 0 1 1-e 0+e 0+e],[0 1 1 1-e 1-e 0+e],c3);plot([0 1 1 0 0],[0 0 1 1 0]);disp('weights');
  "IW{2,1}(134,:)'" : Constant  Value=[-0.328643765864757797512396564343362115323543548583984375;-1.276933252111870586986697162501513957977294921875;1.097953859945065335779190718312747776508331298828125;-1.153794867206221486100048423395492136478424072265625;-1.5442594975204340101981870247982442378997802734375;1.673469912381605251283644975046627223491668701171875;-1.159139076499020593047362126526422798633575439453125;0.1317811894474552880662798770572408102452754974365234375]
      mask Display: e = 0.06;c1 = [120 150 230]/255;c2 = ([120 150 230]+0)/383;c3 = ([120 150 230]+128)/383;patch([0 1 1 0],[0 0 1 1],c1);patch([0 1 1 1-e 1-e 0+e],[0 0 1 1-e 0+e 0+e],c2);patch([0 0 1 1-e 0+e 0+e],[0 1 1 1-e 1-e 0+e],c3);plot([0 1 1 0 0],[0 0 1 1 0]);disp('weights');
  "IW{2,1}(135,:)'" : Constant  Value=[1.4253380172535343728412726704846136271953582763671875;-0.52469999443522008508722365149878896772861480712890625;1.645781957646773374648319077095948159694671630859375;-0.5149944992681885214125259153661318123340606689453125;0.30444887016464150519823306240141391754150390625;-1.5217037329414615509648456281865946948528289794921875;-1.53829529199834968977711469051428139209747314453125;-0.96248226085746335645154658777755685150623321533203125]
      mask Display: e = 0.06;c1 = [120 150 230]/255;c2 = ([120 150 230]+0)/383;c3 = ([120 150 230]+128)/383;patch([0 1 1 0],[0 0 1 1],c1);patch([0 1 1 1-e 1-e 0+e],[0 0 1 1-e 0+e 0+e],c2);patch([0 0 1 1-e 0+e 0+e],[0 1 1 1-e 1-e 0+e],c3);plot([0 1 1 0 0],[0 0 1 1 0]);disp('weights');
  "IW{2,1}(136,:)'" : Constant  Value=[1.8340364443172740838150502895587123930454254150390625;-0.495139273869659890525696255281218327581882476806640625;-1.2288020217730137861877892646589316427707672119140625;1.5993785216609410770871591012110002338886260986328125;-1.2526876259677326430619359598495066165924072265625;0.1816725225549948863346116922912187874317169189453125;-1.287919742756589602805661343154497444629669189453125;-0.12495088404816152849452493001081165857613086700439453125]
      mask Display: e = 0.06;c1 = [120 150 230]/255;c2 = ([120 150 230]+0)/383;c3 = ([120 150 230]+128)/383;patch([0 1 1 0],[0 0 1 1],c1);patch([0 1 1 1-e 1-e 0+e],[0 0 1 1-e 0+e 0+e],c2);patch([0 0 1 1-e 0+e 0+e],[0 1 1 1-e 1-e 0+e],c3);plot([0 1 1 0 0],[0 0 1 1 0]);disp('weights');
  "IW{2,1}(137,:)'" : Constant  Value=[1.2144320976277389600994638385600410401821136474609375;0.53993669110952635659117504474124871194362640380859375;1.7980873460489430470943261752836406230926513671875;-0.1752594036105314945217514832620508968830108642578125;-1.347683724784759728976268888800404965877532958984375;-1.52405694967661187178009640774689614772796630859375;-1.3216497833904288228268342209048569202423095703125;0.2169042246059575962391363646020181477069854736328125]
      mask Display: e = 0.06;c1 = [120 150 230]/255;c2 = ([120 150 230]+0)/383;c3 = ([120 150 230]+128)/383;patch([0 1 1 0],[0 0 1 1],c1);patch([0 1 1 1-e 1-e 0+e],[0 0 1 1-e 0+e 0+e],c2);patch([0 0 1 1-e 0+e 0+e],[0 1 1 1-e 1-e 0+e],c3);plot([0 1 1 0 0],[0 0 1 1 0]);disp('weights');
  "IW{2,1}(138,:)'" : Constant  Value=[1.93517715523273015065797153511084616184234619140625;1.3891910418285957629080940023413859307765960693359375;0.18419004947108608138961471922812052071094512939453125;0.299581378640679074631947287343791685998439788818359375;-1.552318465180493323174459874280728399753570556640625;-1.512560493036712472303406684659421443939208984375;0.59024612509746832156309892525314353406429290771484375;0.399379929496509744613064185614348389208316802978515625]
      mask Display: e = 0.06;c1 = [120 150 230]/255;c2 = ([120 150 230]+0)/383;c3 = ([120 150 230]+128)/383;patch([0 1 1 0],[0 0 1 1],c1);patch([0 1 1 1-e 1-e 0+e],[0 0 1 1-e 0+e 0+e],c2);patch([0 0 1 1-e 0+e 0+e],[0 1 1 1-e 1-e 0+e],c3);plot([0 1 1 0 0],[0 0 1 1 0]);disp('weights');
  "IW{2,1}(139,:)'" : Constant  Value=[0.57025843958936672795090316867572255432605743408203125;0.80125537044495664940058077263529412448406219482421875;-1.723554819950437799747078315704129636287689208984375;-1.3329513871876621511347593695973046123981475830078125;0.7682284175456093322509332210756838321685791015625;-0.9977239525779226791968312682001851499080657958984375;0.11831831034328964269430883859968162141740322113037109375;-1.921530932396787960669826134108006954193115234375]
      mask Display: e = 0.06;c1 = [120 150 230]/255;c2 = ([120 150 230]+0)/383;c3 = ([120 150 230]+128)/383;patch([0 1 1 0],[0 0 1 1],c1);patch([0 1 1 1-e 1-e 0+e],[0 0 1 1-e 0+e 0+e],c2);patch([0 0 1 1-e 0+e 0+e],[0 1 1 1-e 1-e 0+e],c3);plot([0 1 1 0 0],[0 0 1 1 0]);disp('weights');
  "IW{2,1}(14,:)'" : Constant  Value=[-0.1475910918780803104954912896573659963905811309814453125;0.93063732235244500667903366775135509669780731201171875;2.0656724580799874502190505154430866241455078125;-0.8661677990470193488903305478743277490139007568359375;1.6004409232003242724573510713526047766208648681640625;0.989893122394842617239874016377143561840057373046875;1.2498538382076933572761845425702631473541259765625;-0.1300679502076476923289050091625540517270565032958984375]
      mask Display: e = 0.06;c1 = [120 150 230]/255;c2 = ([120 150 230]+0)/383;c3 = ([120 150 230]+128)/383;patch([0 1 1 0],[0 0 1 1],c1);patch([0 1 1 1-e 1-e 0+e],[0 0 1 1-e 0+e 0+e],c2);patch([0 0 1 1-e 0+e 0+e],[0 1 1 1-e 1-e 0+e],c3);plot([0 1 1 0 0],[0 0 1 1 0]);disp('weights');
  "IW{2,1}(140,:)'" : Constant  Value=[-1.1542841193851256509361746793729253113269805908203125;-1.6127651595642518156381584049086086452007293701171875;0.469109486478065218495459021141869015991687774658203125;1.347915997268760879279625441995449364185333251953125;-0.11045948012090746337410251953770057298243045806884765625;-1.258294035940612953794470740831457078456878662109375;-1.081870269578619758732429545489139854907989501953125;1.413113382994770628187097827321849763393402099609375]
      mask Display: e = 0.06;c1 = [120 150 230]/255;c2 = ([120 150 230]+0)/383;c3 = ([120 150 230]+128)/383;patch([0 1 1 0],[0 0 1 1],c1);patch([0 1 1 1-e 1-e 0+e],[0 0 1 1-e 0+e 0+e],c2);patch([0 0 1 1-e 0+e 0+e],[0 1 1 1-e 1-e 0+e],c3);plot([0 1 1 0 0],[0 0 1 1 0]);disp('weights');
  "IW{2,1}(141,:)'" : Constant  Value=[1.555436158116168865461759196477942168712615966796875;1.392645996359309190637532083201222121715545654296875;-1.4485757681466668866931968295830301940441131591796875;-1.1489041357432030476815043584792874753475189208984375;1.357835726053806535418289058725349605083465576171875;-0.74323930565968343575633525688317604362964630126953125;1.012353998766076568216476516681723296642303466796875;0.298658282093629157127878670507925562560558319091796875]
      mask Display: e = 0.06;c1 = [120 150 230]/255;c2 = ([120 150 230]+0)/383;c3 = ([120 150 230]+128)/383;patch([0 1 1 0],[0 0 1 1],c1);patch([0 1 1 1-e 1-e 0+e],[0 0 1 1-e 0+e 0+e],c2);patch([0 0 1 1-e 0+e 0+e],[0 1 1 1-e 1-e 0+e],c3);plot([0 1 1 0 0],[0 0 1 1 0]);disp('weights');
  "IW{2,1}(142,:)'" : Constant  Value=[-1.63648063262928555872122160508297383785247802734375;-0.478335231788780845807451669315923936665058135986328125;0.826940310979516812750489407335408031940460205078125;1.41159101044353807452580440440215170383453369140625;-0.65375268720077650552724435328855179250240325927734375;-0.921157033382365764140331521048210561275482177734375;-1.1070362005738314525871146543067879974842071533203125;1.643424627971423745975698693655431270599365234375]
      mask Display: e = 0.06;c1 = [120 150 230]/255;c2 = ([120 150 230]+0)/383;c3 = ([120 150 230]+128)/383;patch([0 1 1 0],[0 0 1 1],c1);patch([0 1 1 1-e 1-e 0+e],[0 0 1 1-e 0+e 0+e],c2);patch([0 0 1 1-e 0+e 0+e],[0 1 1 1-e 1-e 0+e],c3);plot([0 1 1 0 0],[0 0 1 1 0]);disp('weights');
  "IW{2,1}(143,:)'" : Constant  Value=[-1.5159026996203175396971118971123360097408294677734375;-0.1114566532801510856387494641239754855632781982421875;0.566165381711507986750575582846067845821380615234375;-0.59750212023157944773998906384804286062717437744140625;1.049107503520645412464773471583612263202667236328125;0.81962908610475704307418709504418075084686279296875;1.064366689863233350621385397971607744693756103515625;2.26432122155323423129402726772241294384002685546875]
      mask Display: e = 0.06;c1 = [120 150 230]/255;c2 = ([120 150 230]+0)/383;c3 = ([120 150 230]+128)/383;patch([0 1 1 0],[0 0 1 1],c1);patch([0 1 1 1-e 1-e 0+e],[0 0 1 1-e 0+e 0+e],c2);patch([0 0 1 1-e 0+e 0+e],[0 1 1 1-e 1-e 0+e],c3);plot([0 1 1 0 0],[0 0 1 1 0]);disp('weights');
  "IW{2,1}(144,:)'" : Constant  Value=[1.1393984613578715947568298361147753894329071044921875;-0.26708741927873724808506494809989817440509796142578125;-1.7527699509584000470141518235323019325733184814453125;-0.89396381850880868302766657507163472473621368408203125;-1.2216502601920831150295043698861263692378997802734375;0.02085063011040282077157570483905146829783916473388671875;1.458501559953706117056526636588387191295623779296875;1.48372214129435864293782287859357893466949462890625]
      mask Display: e = 0.06;c1 = [120 150 230]/255;c2 = ([120 150 230]+0)/383;c3 = ([120 150 230]+128)/383;patch([0 1 1 0],[0 0 1 1],c1);patch([0 1 1 1-e 1-e 0+e],[0 0 1 1-e 0+e 0+e],c2);patch([0 0 1 1-e 0+e 0+e],[0 1 1 1-e 1-e 0+e],c3);plot([0 1 1 0 0],[0 0 1 1 0]);disp('weights');
  "IW{2,1}(145,:)'" : Constant  Value=[-1.672498577269726727223542184219695627689361572265625;-0.354042338052804106407478457185789011418819427490234375;-1.5900684986742927851111062409472651779651641845703125;-1.0903594267458378563873111488646827638149261474609375;0.353007963697988425000318102320306934416294097900390625;0.55278986736012125646766435238532721996307373046875;-1.2268092599696480693438616071944124996662139892578125;-1.573885724979420697167142861871980130672454833984375]
      mask Display: e = 0.06;c1 = [120 150 230]/255;c2 = ([120 150 230]+0)/383;c3 = ([120 150 230]+128)/383;patch([0 1 1 0],[0 0 1 1],c1);patch([0 1 1 1-e 1-e 0+e],[0 0 1 1-e 0+e 0+e],c2);patch([0 0 1 1-e 0+e 0+e],[0 1 1 1-e 1-e 0+e],c3);plot([0 1 1 0 0],[0 0 1 1 0]);disp('weights');
  "IW{2,1}(146,:)'" : Constant  Value=[0.179595391227207412665478614144376479089260101318359375;0.0147496024470601984346362911537653417326509952545166015625;-1.0560776403535425682633785982034169137477874755859375;-1.6969323856982783116364998932112939655780792236328125;1.6828198583554636602599430261761881411075592041015625;0.5509684967733530225331151086720637977123260498046875;1.4080465532479335966087319320649839937686920166015625;-1.0568011535181851545672770953387953341007232666015625]
      mask Display: e = 0.06;c1 = [120 150 230]/255;c2 = ([120 150 230]+0)/383;c3 = ([120 150 230]+128)/383;patch([0 1 1 0],[0 0 1 1],c1);patch([0 1 1 1-e 1-e 0+e],[0 0 1 1-e 0+e 0+e],c2);patch([0 0 1 1-e 0+e 0+e],[0 1 1 1-e 1-e 0+e],c3);plot([0 1 1 0 0],[0 0 1 1 0]);disp('weights');
  "IW{2,1}(147,:)'" : Constant  Value=[-1.03132267851302827921244897879660129547119140625;1.550328661952410147506498105940409004688262939453125;-0.311524372001474814108945565749309025704860687255859375;-1.18458407133541765432482861797325313091278076171875;0.311784068302015715534736273184535093605518341064453125;-0.6412131706496195793221204439760185778141021728515625;1.9770601597342498667586596639011986553668975830078125;-1.2466773160082496030298671030323021113872528076171875]
      mask Display: e = 0.06;c1 = [120 150 230]/255;c2 = ([120 150 230]+0)/383;c3 = ([120 150 230]+128)/383;patch([0 1 1 0],[0 0 1 1],c1);patch([0 1 1 1-e 1-e 0+e],[0 0 1 1-e 0+e 0+e],c2);patch([0 0 1 1-e 0+e 0+e],[0 1 1 1-e 1-e 0+e],c3);plot([0 1 1 0 0],[0 0 1 1 0]);disp('weights');
  "IW{2,1}(148,:)'" : Constant  Value=[-0.054493161846729941399924967981860390864312648773193359375;0.5343676154032148684080993916722945868968963623046875;-1.473090610177091974719587597064673900604248046875;1.0271244177301923627965152263641357421875;1.49656463137482464986760533065535128116607666015625;1.23872433238006163236377688008360564708709716796875;-1.4886462264960254042733822643640451133251190185546875;1.2380635596750291238521413106354884803295135498046875]
      mask Display: e = 0.06;c1 = [120 150 230]/255;c2 = ([120 150 230]+0)/383;c3 = ([120 150 230]+128)/383;patch([0 1 1 0],[0 0 1 1],c1);patch([0 1 1 1-e 1-e 0+e],[0 0 1 1-e 0+e 0+e],c2);patch([0 0 1 1-e 0+e 0+e],[0 1 1 1-e 1-e 0+e],c3);plot([0 1 1 0 0],[0 0 1 1 0]);disp('weights');
  "IW{2,1}(149,:)'" : Constant  Value=[-0.58871923307587958884568024586769752204418182373046875;-0.7157862723880208388749224468483589589595794677734375;1.95900745794487374240588906104676425457000732421875;0.82905205768125844745242147837416268885135650634765625;-0.36761722384331563251436136852134950459003448486328125;0.2367872792273712223565240719835855998098850250244140625;1.7618670638451929821854946567327715456485748291015625;-1.495211735856859291970977210439741611480712890625]
      mask Display: e = 0.06;c1 = [120 150 230]/255;c2 = ([120 150 230]+0)/383;c3 = ([120 150 230]+128)/383;patch([0 1 1 0],[0 0 1 1],c1);patch([0 1 1 1-e 1-e 0+e],[0 0 1 1-e 0+e 0+e],c2);patch([0 0 1 1-e 0+e 0+e],[0 1 1 1-e 1-e 0+e],c3);plot([0 1 1 0 0],[0 0 1 1 0]);disp('weights');
  "IW{2,1}(15,:)'" : Constant  Value=[-0.08642998162410982232461975627302308566868305206298828125;1.564054504705512105289244573214091360569000244140625;-1.9530986638336447214214786072261631488800048828125;-1.2038894069802894559728656531660817563533782958984375;0.16752361741504906422761678186361677944660186767578125;-0.52443506654011429191086790524423122406005859375;1.6088197415876377416310560874990187585353851318359375;-0.67999581746761805778334064598311670124530792236328125]
      mask Display: e = 0.06;c1 = [120 150 230]/255;c2 = ([120 150 230]+0)/383;c3 = ([120 150 230]+128)/383;patch([0 1 1 0],[0 0 1 1],c1);patch([0 1 1 1-e 1-e 0+e],[0 0 1 1-e 0+e 0+e],c2);patch([0 0 1 1-e 0+e 0+e],[0 1 1 1-e 1-e 0+e],c3);plot([0 1 1 0 0],[0 0 1 1 0]);disp('weights');
  "IW{2,1}(150,:)'" : Constant  Value=[1.4728445482729257687282142796902917325496673583984375;0.449501207629826760037161648142500780522823333740234375;-0.7271880415471028147322840595734305679798126220703125;1.8810654481322834907786045732791535556316375732421875;-0.672529075612093851788131360081024467945098876953125;-1.486131027607958454694880856550298631191253662109375;1.4767325229975114542213532331516034901142120361328125;0.1254705705667645554424183274022652767598628997802734375]
      mask Display: e = 0.06;c1 = [120 150 230]/255;c2 = ([120 150 230]+0)/383;c3 = ([120 150 230]+128)/383;patch([0 1 1 0],[0 0 1 1],c1);patch([0 1 1 1-e 1-e 0+e],[0 0 1 1-e 0+e 0+e],c2);patch([0 0 1 1-e 0+e 0+e],[0 1 1 1-e 1-e 0+e],c3);plot([0 1 1 0 0],[0 0 1 1 0]);disp('weights');
  "IW{2,1}(151,:)'" : Constant  Value=[0.474883185258799966899090350125334225594997406005859375;-0.94811705894487141588200529440655373036861419677734375;1.8949961130196621983401428224169649183750152587890625;1.9304969966867233654994606695254333317279815673828125;-0.2337314744018714474105280487492564134299755096435546875;1.0044661622643340503913123029633425176143646240234375;-0.6367709514460579978134546763612888753414154052734375;-1.0446189268810364136896851050551049411296844482421875]
      mask Display: e = 0.06;c1 = [120 150 230]/255;c2 = ([120 150 230]+0)/383;c3 = ([120 150 230]+128)/383;patch([0 1 1 0],[0 0 1 1],c1);patch([0 1 1 1-e 1-e 0+e],[0 0 1 1-e 0+e 0+e],c2);patch([0 0 1 1-e 0+e 0+e],[0 1 1 1-e 1-e 0+e],c3);plot([0 1 1 0 0],[0 0 1 1 0]);disp('weights');
  "IW{2,1}(152,:)'" : Constant  Value=[1.7971482360408626011150090562296099960803985595703125;0.1556846188495674965235338049751590006053447723388671875;-0.2376049707330309679331747929609264247119426727294921875;-1.0394033348376101599797038943506777286529541015625;1.4810573947868646005332493587047792971134185791015625;-1.10125674259872052829223321168683469295501708984375;1.697171605917245695849260300747118890285491943359375;0.48528843537099219940245120596955530345439910888671875]
      mask Display: e = 0.06;c1 = [120 150 230]/255;c2 = ([120 150 230]+0)/383;c3 = ([120 150 230]+128)/383;patch([0 1 1 0],[0 0 1 1],c1);patch([0 1 1 1-e 1-e 0+e],[0 0 1 1-e 0+e 0+e],c2);patch([0 0 1 1-e 0+e 0+e],[0 1 1 1-e 1-e 0+e],c3);plot([0 1 1 0 0],[0 0 1 1 0]);disp('weights');
  "IW{2,1}(153,:)'" : Constant  Value=[0.354410973899148384891333307677996344864368438720703125;-0.89010302286270304161774902240722440183162689208984375;1.5646326148445464099268065183423459529876708984375;-0.98269665320951649079006529063917696475982666015625;1.3436082797800821264644355323980562388896942138671875;-1.003937431537902824629782116971909999847412109375;-0.9878489312368732289115769162890501320362091064453125;-1.7080466612864089182011184675502590835094451904296875]
      mask Display: e = 0.06;c1 = [120 150 230]/255;c2 = ([120 150 230]+0)/383;c3 = ([120 150 230]+128)/383;patch([0 1 1 0],[0 0 1 1],c1);patch([0 1 1 1-e 1-e 0+e],[0 0 1 1-e 0+e 0+e],c2);patch([0 0 1 1-e 0+e 0+e],[0 1 1 1-e 1-e 0+e],c3);plot([0 1 1 0 0],[0 0 1 1 0]);disp('weights');
  "IW{2,1}(154,:)'" : Constant  Value=[0.479333280429032004832379243453033268451690673828125;-0.324652519229142455525760624368558637797832489013671875;1.454094275409585801384082515141926705837249755859375;1.3949174751412254380511512863449752330780029296875;0.78989456480209885302912198312697000801563262939453125;1.5344667056307115249325079275877214968204498291015625;1.2507596545847230462555899066501297056674957275390625;-1.4609573844773520168160985122085548937320709228515625]
      mask Display: e = 0.06;c1 = [120 150 230]/255;c2 = ([120 150 230]+0)/383;c3 = ([120 150 230]+128)/383;patch([0 1 1 0],[0 0 1 1],c1);patch([0 1 1 1-e 1-e 0+e],[0 0 1 1-e 0+e 0+e],c2);patch([0 0 1 1-e 0+e 0+e],[0 1 1 1-e 1-e 0+e],c3);plot([0 1 1 0 0],[0 0 1 1 0]);disp('weights');
  "IW{2,1}(155,:)'" : Constant  Value=[2.00289540303800439602355254464782774448394775390625;-1.56085702789567104531442964798770844936370849609375;-0.7064379031930976271524968979065306484699249267578125;0.7691686717439980558452816694625653326511383056640625;1.185735636351793242937446848372928798198699951171875;-0.7797081013718223374553417670540511608123779296875;-1.190014911816073439609908746206201612949371337890625;0.424442939152618825549012626652256585657596588134765625]
      mask Display: e = 0.06;c1 = [120 150 230]/255;c2 = ([120 150 230]+0)/383;c3 = ([120 150 230]+128)/383;patch([0 1 1 0],[0 0 1 1],c1);patch([0 1 1 1-e 1-e 0+e],[0 0 1 1-e 0+e 0+e],c2);patch([0 0 1 1-e 0+e 0+e],[0 1 1 1-e 1-e 0+e],c3);plot([0 1 1 0 0],[0 0 1 1 0]);disp('weights');
  "IW{2,1}(156,:)'" : Constant  Value=[1.094947012688101128929929473088122904300689697265625;0.903505344105733687598558390163816511631011962890625;-1.82186430760528050853963577537797391414642333984375;1.7625773911467323973312204543617554008960723876953125;-1.0731563285242966543364673270843923091888427734375;-0.4361825280718887309916453887126408517360687255859375;-1.1311764865781934741306713476660661399364471435546875;-0.18845489687891703312061508768238127231597900390625]
      mask Display: e = 0.06;c1 = [120 150 230]/255;c2 = ([120 150 230]+0)/383;c3 = ([120 150 230]+128)/383;patch([0 1 1 0],[0 0 1 1],c1);patch([0 1 1 1-e 1-e 0+e],[0 0 1 1-e 0+e 0+e],c2);patch([0 0 1 1-e 0+e 0+e],[0 1 1 1-e 1-e 0+e],c3);plot([0 1 1 0 0],[0 0 1 1 0]);disp('weights');
  "IW{2,1}(157,:)'" : Constant  Value=[-1.4656515050783374132237213416374288499355316162109375;1.47114512421566967503849809872917830944061279296875;-1.7988716528416708317905658987001515924930572509765625;-1.0661402235700183638300586608238518238067626953125;-0.007442376242258908793092420097536887624301016330718994140625;-1.188494756144137465270205211709253489971160888671875;0.67591817498625328397565681370906531810760498046875;0.489772640075894993838545588005217723548412322998046875]
      mask Display: e = 0.06;c1 = [120 150 230]/255;c2 = ([120 150 230]+0)/383;c3 = ([120 150 230]+128)/383;patch([0 1 1 0],[0 0 1 1],c1);patch([0 1 1 1-e 1-e 0+e],[0 0 1 1-e 0+e 0+e],c2);patch([0 0 1 1-e 0+e 0+e],[0 1 1 1-e 1-e 0+e],c3);plot([0 1 1 0 0],[0 0 1 1 0]);disp('weights');
  "IW{2,1}(158,:)'" : Constant  Value=[1.2448115001294777215434805839322507381439208984375;-1.48595248767241283616158398217521607875823974609375;1.3573311340308062966641955426894128322601318359375;1.4395633752923888692976106540299952030181884765625;1.215655396665385357124478105106391012668609619140625;0.09807998447919218099055882476022816263139247894287109375;0.5425822555173487327095926957554183900356292724609375;-1.317725994508947451322455890476703643798828125]
      mask Display: e = 0.06;c1 = [120 150 230]/255;c2 = ([120 150 230]+0)/383;c3 = ([120 150 230]+128)/383;patch([0 1 1 0],[0 0 1 1],c1);patch([0 1 1 1-e 1-e 0+e],[0 0 1 1-e 0+e 0+e],c2);patch([0 0 1 1-e 0+e 0+e],[0 1 1 1-e 1-e 0+e],c3);plot([0 1 1 0 0],[0 0 1 1 0]);disp('weights');
  "IW{2,1}(159,:)'" : Constant  Value=[-1.06910762514044055393469534465111792087554931640625;1.0695006404979505720831411963445134460926055908203125;-0.9800227127228591239571642290684394538402557373046875;-1.434321577868478581052613662905059754848480224609375;1.455182321473289075441925888299010694026947021484375;-0.031712214758177238727032687393148080445826053619384765625;1.5941993792256254902639511783490888774394989013671875;1.0247776161367314617933743647881783545017242431640625]
      mask Display: e = 0.06;c1 = [120 150 230]/255;c2 = ([120 150 230]+0)/383;c3 = ([120 150 230]+128)/383;patch([0 1 1 0],[0 0 1 1],c1);patch([0 1 1 1-e 1-e 0+e],[0 0 1 1-e 0+e 0+e],c2);patch([0 0 1 1-e 0+e 0+e],[0 1 1 1-e 1-e 0+e],c3);plot([0 1 1 0 0],[0 0 1 1 0]);disp('weights');
  "IW{2,1}(16,:)'" : Constant  Value=[1.5280592480067538563304196941317059099674224853515625;0.705876981432926431381247311946935951709747314453125;-2.213087813991118313339256928884424269199371337890625;0.204809717915754807560091421692050062119960784912109375;0.398245622952119904258694305099197663366794586181640625;-0.78581339666398519749890283492277376353740692138671875;-1.4031340290128075931619378025061450898647308349609375;-0.6824711884687264529247840982861816883087158203125]
      mask Display: e = 0.06;c1 = [120 150 230]/255;c2 = ([120 150 230]+0)/383;c3 = ([120 150 230]+128)/383;patch([0 1 1 0],[0 0 1 1],c1);patch([0 1 1 1-e 1-e 0+e],[0 0 1 1-e 0+e 0+e],c2);patch([0 0 1 1-e 0+e 0+e],[0 1 1 1-e 1-e 0+e],c3);plot([0 1 1 0 0],[0 0 1 1 0]);disp('weights');
  "IW{2,1}(160,:)'" : Constant  Value=[0.1479821651356516276631936079866136424243450164794921875;1.7088913453732736957846327641163952648639678955078125;-1.973912184023610461025555196101777255535125732421875;0.7004078777758502294403797350241802632808685302734375;0.427804085265997058318276913269073702394962310791015625;-0.9434937920785391174405276615289039909839630126953125;-1.6262412522389404490041897588525898754596710205078125;-0.139386024024501342655213420584914274513721466064453125]
      mask Display: e = 0.06;c1 = [120 150 230]/255;c2 = ([120 150 230]+0)/383;c3 = ([120 150 230]+128)/383;patch([0 1 1 0],[0 0 1 1],c1);patch([0 1 1 1-e 1-e 0+e],[0 0 1 1-e 0+e 0+e],c2);patch([0 0 1 1-e 0+e 0+e],[0 1 1 1-e 1-e 0+e],c3);plot([0 1 1 0 0],[0 0 1 1 0]);disp('weights');
  "IW{2,1}(161,:)'" : Constant  Value=[-2.575482700333208807563778464100323617458343505859375;0.4345760548802932721201841559377498924732208251953125;-0.347718926366610003864110467475256882607936859130859375;0.544220248462720324056363097042776644229888916015625;0.7834355102295973427573017033864744007587432861328125;-1.3915543547789319678287256465409882366657257080078125;-1.0451619119446100558690204707090742886066436767578125;-0.489052598245619363215297425995231606066226959228515625]
      mask Display: e = 0.06;c1 = [120 150 230]/255;c2 = ([120 150 230]+0)/383;c3 = ([120 150 230]+128)/383;patch([0 1 1 0],[0 0 1 1],c1);patch([0 1 1 1-e 1-e 0+e],[0 0 1 1-e 0+e 0+e],c2);patch([0 0 1 1-e 0+e 0+e],[0 1 1 1-e 1-e 0+e],c3);plot([0 1 1 0 0],[0 0 1 1 0]);disp('weights');
  "IW{2,1}(162,:)'" : Constant  Value=[1.113230805895442987463184181251563131809234619140625;-1.1648692497588786221029977241414599120616912841796875;-0.6950354630741542028005142128677107393741607666015625;0.98983596212279412185353066888637840747833251953125;-0.86368203308301760845466787941404618322849273681640625;1.3475339886785473453301165136508643627166748046875;-1.3054390176527892464264368754811584949493408203125;1.654199390438355177224138969904743134975433349609375]
      mask Display: e = 0.06;c1 = [120 150 230]/255;c2 = ([120 150 230]+0)/383;c3 = ([120 150 230]+128)/383;patch([0 1 1 0],[0 0 1 1],c1);patch([0 1 1 1-e 1-e 0+e],[0 0 1 1-e 0+e 0+e],c2);patch([0 0 1 1-e 0+e 0+e],[0 1 1 1-e 1-e 0+e],c3);plot([0 1 1 0 0],[0 0 1 1 0]);disp('weights');
  "IW{2,1}(163,:)'" : Constant  Value=[-0.8663140553212347327871611923910677433013916015625;1.1999988292001908529726961205597035586833953857421875;-0.464779851309625124944346907795988954603672027587890625;2.50077904405880868665690286434255540370941162109375;-0.488869907693681382543360314230085350573062896728515625;-1.373557404508769508311161189340054988861083984375;-0.497969998583333239849935125675983726978302001953125;0.236084588594673683292768373576109297573566436767578125]
      mask Display: e = 0.06;c1 = [120 150 230]/255;c2 = ([120 150 230]+0)/383;c3 = ([120 150 230]+128)/383;patch([0 1 1 0],[0 0 1 1],c1);patch([0 1 1 1-e 1-e 0+e],[0 0 1 1-e 0+e 0+e],c2);patch([0 0 1 1-e 0+e 0+e],[0 1 1 1-e 1-e 0+e],c3);plot([0 1 1 0 0],[0 0 1 1 0]);disp('weights');
  "IW{2,1}(164,:)'" : Constant  Value=[0.167201587435335585762885557414847426116466522216796875;-1.3116135935789288158304088938166387379169464111328125;1.6592460502091490592846412255312316119670867919921875;-1.69866610856499988813084200955927371978759765625;-0.7371453700955175047937473209458403289318084716796875;-0.482997364410623741814987397447112016379833221435546875;0.74789092122008227203622254819492809474468231201171875;1.5210041484928513710883635212667286396026611328125]
      mask Display: e = 0.06;c1 = [120 150 230]/255;c2 = ([120 150 230]+0)/383;c3 = ([120 150 230]+128)/383;patch([0 1 1 0],[0 0 1 1],c1);patch([0 1 1 1-e 1-e 0+e],[0 0 1 1-e 0+e 0+e],c2);patch([0 0 1 1-e 0+e 0+e],[0 1 1 1-e 1-e 0+e],c3);plot([0 1 1 0 0],[0 0 1 1 0]);disp('weights');
  "IW{2,1}(165,:)'" : Constant  Value=[-0.218268899220343925993148559427936561405658721923828125;-0.7219191170099943377636009245179593563079833984375;-0.9834995997412281365512853881227783858776092529296875;-0.77985028653635291018275665919645689427852630615234375;0.50958938454644542304095011786557734012603759765625;1.3666764448696400169325215756543911993503570556640625;-1.30369803194212874331014972995035350322723388671875;2.183240455141489899659745788085274398326873779296875]
      mask Display: e = 0.06;c1 = [120 150 230]/255;c2 = ([120 150 230]+0)/383;c3 = ([120 150 230]+128)/383;patch([0 1 1 0],[0 0 1 1],c1);patch([0 1 1 1-e 1-e 0+e],[0 0 1 1-e 0+e 0+e],c2);patch([0 0 1 1-e 0+e 0+e],[0 1 1 1-e 1-e 0+e],c3);plot([0 1 1 0 0],[0 0 1 1 0]);disp('weights');
  "IW{2,1}(166,:)'" : Constant  Value=[0.98325283558789389193321994753205217421054840087890625;-0.97977592210045749698821282436256296932697296142578125;1.2965725339675981953035943661234341561794281005859375;-0.2428079863357864021100596119140391238033771514892578125;-1.9033537731749616828125226675183512270450592041015625;1.148450705770631241620094442623667418956756591796875;0.79646256900773970688334202350233681499958038330078125;-1.3124292669733359506523129311972297728061676025390625]
      mask Display: e = 0.06;c1 = [120 150 230]/255;c2 = ([120 150 230]+0)/383;c3 = ([120 150 230]+128)/383;patch([0 1 1 0],[0 0 1 1],c1);patch([0 1 1 1-e 1-e 0+e],[0 0 1 1-e 0+e 0+e],c2);patch([0 0 1 1-e 0+e 0+e],[0 1 1 1-e 1-e 0+e],c3);plot([0 1 1 0 0],[0 0 1 1 0]);disp('weights');
  "IW{2,1}(167,:)'" : Constant  Value=[-1.4025207869228670798378288964158855378627777099609375;0.377511248815475874973657255395664833486080169677734375;-1.505128082642681608405155202490277588367462158203125;-0.07472585569521682236082682493361062370240688323974609375;-0.80576020598713882225894167277147062122821807861328125;-1.52532793120149090526638246956281363964080810546875;2.014097226715455324352888055727817118167877197265625;0.1736465192820394742856393577312701381742954254150390625]
      mask Display: e = 0.06;c1 = [120 150 230]/255;c2 = ([120 150 230]+0)/383;c3 = ([120 150 230]+128)/383;patch([0 1 1 0],[0 0 1 1],c1);patch([0 1 1 1-e 1-e 0+e],[0 0 1 1-e 0+e 0+e],c2);patch([0 0 1 1-e 0+e 0+e],[0 1 1 1-e 1-e 0+e],c3);plot([0 1 1 0 0],[0 0 1 1 0]);disp('weights');
  "IW{2,1}(168,:)'" : Constant  Value=[-2.275606893311238110300109838135540485382080078125;-0.76370070310602222729556842750753276050090789794921875;-0.9473417580959260231310281596961431205272674560546875;0.1734720203278311279060375227345502935349941253662109375;-0.39428383412900480653462409463827498257160186767578125;1.445635354300652597459020398673601448535919189453125;-1.29273789098291569388265997986309230327606201171875;-0.57689914127338060012561982148326933383941650390625]
      mask Display: e = 0.06;c1 = [120 150 230]/255;c2 = ([120 150 230]+0)/383;c3 = ([120 150 230]+128)/383;patch([0 1 1 0],[0 0 1 1],c1);patch([0 1 1 1-e 1-e 0+e],[0 0 1 1-e 0+e 0+e],c2);patch([0 0 1 1-e 0+e 0+e],[0 1 1 1-e 1-e 0+e],c3);plot([0 1 1 0 0],[0 0 1 1 0]);disp('weights');
  "IW{2,1}(169,:)'" : Constant  Value=[-0.449570052188346058752443923367536626756191253662109375;-0.476531315675093825046104711873340420424938201904296875;0.894005438648663552925199837773106992244720458984375;-1.9005271925430291535263904734165407717227935791015625;-0.9473525039608838849147787186666391789913177490234375;0.34796127710326008042329704039730131626129150390625;-1.8714364809585501969735332750133238732814788818359375;-1.2695877967387685369970995452604256570339202880859375]
      mask Display: e = 0.06;c1 = [120 150 230]/255;c2 = ([120 150 230]+0)/383;c3 = ([120 150 230]+128)/383;patch([0 1 1 0],[0 0 1 1],c1);patch([0 1 1 1-e 1-e 0+e],[0 0 1 1-e 0+e 0+e],c2);patch([0 0 1 1-e 0+e 0+e],[0 1 1 1-e 1-e 0+e],c3);plot([0 1 1 0 0],[0 0 1 1 0]);disp('weights');
  "IW{2,1}(17,:)'" : Constant  Value=[-0.1288381436509566935200155057827942073345184326171875;1.60040277450735946018767208443023264408111572265625;-1.0513488782393007880955337896011769771575927734375;1.0529837263559291837822229354060254991054534912109375;1.8232078675512923826573796759475953876972198486328125;-1.3951211478220406636552297641173936426639556884765625;0.97470111633032552322930541777168400585651397705078125;0.08834127717385402422944906675184029154479503631591796875]
      mask Display: e = 0.06;c1 = [120 150 230]/255;c2 = ([120 150 230]+0)/383;c3 = ([120 150 230]+128)/383;patch([0 1 1 0],[0 0 1 1],c1);patch([0 1 1 1-e 1-e 0+e],[0 0 1 1-e 0+e 0+e],c2);patch([0 0 1 1-e 0+e 0+e],[0 1 1 1-e 1-e 0+e],c3);plot([0 1 1 0 0],[0 0 1 1 0]);disp('weights');
  "IW{2,1}(170,:)'" : Constant  Value=[-1.3476953979017214368951727010426111519336700439453125;1.649320513597154036489200734649784862995147705078125;-0.475705215839788919662822763712028972804546356201171875;0.91402785518355045280003423613379709422588348388671875;-1.428409015630015321818291340605355799198150634765625;1.73109535883129073141617482178844511508941650390625;0.49570054073123792637289852791582234203815460205078125;-0.360233738417770954498564606183208525180816650390625]
      mask Display: e = 0.06;c1 = [120 150 230]/255;c2 = ([120 150 230]+0)/383;c3 = ([120 150 230]+128)/383;patch([0 1 1 0],[0 0 1 1],c1);patch([0 1 1 1-e 1-e 0+e],[0 0 1 1-e 0+e 0+e],c2);patch([0 0 1 1-e 0+e 0+e],[0 1 1 1-e 1-e 0+e],c3);plot([0 1 1 0 0],[0 0 1 1 0]);disp('weights');
  "IW{2,1}(171,:)'" : Constant  Value=[-1.45400037200095599843052696087397634983062744140625;-0.1959274512625721331726680318752187304198741912841796875;1.5683753167350198420848528257920406758785247802734375;-1.788508551632197463021611838485114276409149169921875;0.649269531934987043086948688142001628875732421875;0.38131966155556240583024418810964561998844146728515625;1.09432423866136208090438231010921299457550048828125;-1.231850770574885789443442263291217386722564697265625]
      mask Display: e = 0.06;c1 = [120 150 230]/255;c2 = ([120 150 230]+0)/383;c3 = ([120 150 230]+128)/383;patch([0 1 1 0],[0 0 1 1],c1);patch([0 1 1 1-e 1-e 0+e],[0 0 1 1-e 0+e 0+e],c2);patch([0 0 1 1-e 0+e 0+e],[0 1 1 1-e 1-e 0+e],c3);plot([0 1 1 0 0],[0 0 1 1 0]);disp('weights');
  "IW{2,1}(172,:)'" : Constant  Value=[1.3574614882023972040059334176476113498210906982421875;1.0710556543439928578465014652465470135211944580078125;1.53610748955831777351477285264991223812103271484375;1.1868853563452328447880290696048177778720855712890625;-0.581575342472053780085161633905954658985137939453125;1.1238665615911085371436683999490924179553985595703125;0.463685184074650258434502347881789319217205047607421875;1.54368807396102969420326189720071852207183837890625]
      mask Display: e = 0.06;c1 = [120 150 230]/255;c2 = ([120 150 230]+0)/383;c3 = ([120 150 230]+128)/383;patch([0 1 1 0],[0 0 1 1],c1);patch([0 1 1 1-e 1-e 0+e],[0 0 1 1-e 0+e 0+e],c2);patch([0 0 1 1-e 0+e 0+e],[0 1 1 1-e 1-e 0+e],c3);plot([0 1 1 0 0],[0 0 1 1 0]);disp('weights');
  "IW{2,1}(173,:)'" : Constant  Value=[-0.70318908734606921928644851504941470921039581298828125;-0.266232605001410382872251148000941611826419830322265625;-1.9132436859050814259575190590112470090389251708984375;-0.094879511963208151836823844860191456973552703857421875;-0.972525988183672307485494457068853080272674560546875;-1.1837848934346852924903714665560983121395111083984375;-1.24750022545018079966894219978712499141693115234375;1.6652275283860096255494909200933761894702911376953125]
      mask Display: e = 0.06;c1 = [120 150 230]/255;c2 = ([120 150 230]+0)/383;c3 = ([120 150 230]+128)/383;patch([0 1 1 0],[0 0 1 1],c1);patch([0 1 1 1-e 1-e 0+e],[0 0 1 1-e 0+e 0+e],c2);patch([0 0 1 1-e 0+e 0+e],[0 1 1 1-e 1-e 0+e],c3);plot([0 1 1 0 0],[0 0 1 1 0]);disp('weights');
  "IW{2,1}(174,:)'" : Constant  Value=[1.233709795693186617171477337251417338848114013671875;1.3600632481945240659371165747870691120624542236328125;0.62212865461304678316167837692773900926113128662109375;-0.218379064664079691748810319040785543620586395263671875;-1.242559116550491893349317251704633235931396484375;1.0320041356132356735741950615192763507366180419921875;-1.2334341359766243240159155902802012860774993896484375;-1.7118009586359110851816467402386479079723358154296875]
      mask Display: e = 0.06;c1 = [120 150 230]/255;c2 = ([120 150 230]+0)/383;c3 = ([120 150 230]+128)/383;patch([0 1 1 0],[0 0 1 1],c1);patch([0 1 1 1-e 1-e 0+e],[0 0 1 1-e 0+e 0+e],c2);patch([0 0 1 1-e 0+e 0+e],[0 1 1 1-e 1-e 0+e],c3);plot([0 1 1 0 0],[0 0 1 1 0]);disp('weights');
  "IW{2,1}(175,:)'" : Constant  Value=[1.3352042203128231534492442733608186244964599609375;0.93019845004116274989058865685365162789821624755859375;1.3482301283672806224700480015599168837070465087890625;-1.046079395164466685486104324809275567531585693359375;0.01504093975139317827804941174463237985037267208099365234375;-1.5681674402021978931287549130502156913280487060546875;-1.449239781346078448365233271033503115177154541015625;0.8817942948800576719037280781776644289493560791015625]
      mask Display: e = 0.06;c1 = [120 150 230]/255;c2 = ([120 150 230]+0)/383;c3 = ([120 150 230]+128)/383;patch([0 1 1 0],[0 0 1 1],c1);patch([0 1 1 1-e 1-e 0+e],[0 0 1 1-e 0+e 0+e],c2);patch([0 0 1 1-e 0+e 0+e],[0 1 1 1-e 1-e 0+e],c3);plot([0 1 1 0 0],[0 0 1 1 0]);disp('weights');
  "IW{2,1}(176,:)'" : Constant  Value=[0.97068385902106424367730141966603696346282958984375;-1.1620859634256774928218192144413478672504425048828125;1.484306362095933362610367112210951745510101318359375;-0.9455617615265230480048330719000659883022308349609375;-1.465190078093863146335706915124319493770599365234375;-1.35093107320681848904087019036523997783660888671875;0.97042545911064304053894602475338615477085113525390625;-0.82999412889975399121311738781514577567577362060546875]
      mask Display: e = 0.06;c1 = [120 150 230]/255;c2 = ([120 150 230]+0)/383;c3 = ([120 150 230]+128)/383;patch([0 1 1 0],[0 0 1 1],c1);patch([0 1 1 1-e 1-e 0+e],[0 0 1 1-e 0+e 0+e],c2);patch([0 0 1 1-e 0+e 0+e],[0 1 1 1-e 1-e 0+e],c3);plot([0 1 1 0 0],[0 0 1 1 0]);disp('weights');
  "IW{2,1}(177,:)'" : Constant  Value=[1.4908170504009976564674389010178856551647186279296875;-0.98365662123472452638139884584234096109867095947265625;0.330451644562491153589434134119073860347270965576171875;0.851298684071292388608753753942437469959259033203125;0.12532162659246892655318106335471384227275848388671875;2.184429131703858661950334862922318279743194580078125;1.1342518745197491814025170242530293762683868408203125;-0.9965802114933264288509917605551891028881072998046875]
      mask Display: e = 0.06;c1 = [120 150 230]/255;c2 = ([120 150 230]+0)/383;c3 = ([120 150 230]+128)/383;patch([0 1 1 0],[0 0 1 1],c1);patch([0 1 1 1-e 1-e 0+e],[0 0 1 1-e 0+e 0+e],c2);patch([0 0 1 1-e 0+e 0+e],[0 1 1 1-e 1-e 0+e],c3);plot([0 1 1 0 0],[0 0 1 1 0]);disp('weights');
  "IW{2,1}(178,:)'" : Constant  Value=[1.6565413967675557405101471886155195534229278564453125;1.183494058534602988430606274050660431385040283203125;-0.315111938753271314528348057137918658554553985595703125;0.6774403003798987743522275195573456585407257080078125;0.83226857675990262297460731133469380438327789306640625;1.4340576394766724188656326077762059867382049560546875;-1.80238353993089805982208417844958603382110595703125;-0.78251286672653208587036033350159414112567901611328125]
      mask Display: e = 0.06;c1 = [120 150 230]/255;c2 = ([120 150 230]+0)/383;c3 = ([120 150 230]+128)/383;patch([0 1 1 0],[0 0 1 1],c1);patch([0 1 1 1-e 1-e 0+e],[0 0 1 1-e 0+e 0+e],c2);patch([0 0 1 1-e 0+e 0+e],[0 1 1 1-e 1-e 0+e],c3);plot([0 1 1 0 0],[0 0 1 1 0]);disp('weights');
  "IW{2,1}(179,:)'" : Constant  Value=[0.065311797553269601568359803422936238348484039306640625;-1.2352909623413264039726300325128249824047088623046875;0.52539109599824762586450788148795254528522491455078125;-0.1761409487024371001151479276813915930688381195068359375;0.54343335022649641441461199065088294446468353271484375;1.7427583739624525893674444887437857687473297119140625;1.5484147171067081938389264905708841979503631591796875;1.8508168891202725347966406843625009059906005859375]
      mask Display: e = 0.06;c1 = [120 150 230]/255;c2 = ([120 150 230]+0)/383;c3 = ([120 150 230]+128)/383;patch([0 1 1 0],[0 0 1 1],c1);patch([0 1 1 1-e 1-e 0+e],[0 0 1 1-e 0+e 0+e],c2);patch([0 0 1 1-e 0+e 0+e],[0 1 1 1-e 1-e 0+e],c3);plot([0 1 1 0 0],[0 0 1 1 0]);disp('weights');
  "IW{2,1}(18,:)'" : Constant  Value=[-0.722799401796281326681992140947841107845306396484375;-0.840503723715797956828055248479358851909637451171875;-0.283004926468522655103043916824390180408954620361328125;0.446180766261637717917665213462896645069122314453125;0.6475246501013971478499797740369103848934173583984375;1.28754007731695008232009058701805770397186279296875;2.27472018838142542307423354941420257091522216796875;-1.506311921105454754155061891651712357997894287109375]
      mask Display: e = 0.06;c1 = [120 150 230]/255;c2 = ([120 150 230]+0)/383;c3 = ([120 150 230]+128)/383;patch([0 1 1 0],[0 0 1 1],c1);patch([0 1 1 1-e 1-e 0+e],[0 0 1 1-e 0+e 0+e],c2);patch([0 0 1 1-e 0+e 0+e],[0 1 1 1-e 1-e 0+e],c3);plot([0 1 1 0 0],[0 0 1 1 0]);disp('weights');
  "IW{2,1}(180,:)'" : Constant  Value=[1.0041122239771678170683344433200545608997344970703125;-1.3048711219564153029892850099713541567325592041015625;-0.941933849927353517017536432831548154354095458984375;0.6275283169538727889857909758575260639190673828125;1.886447288675902722587807147647254168987274169921875;1.0144795094583496375406639344873838126659393310546875;1.5750050864551587981310376562760211527347564697265625;0.054124516042379881841650757223760592751204967498779296875]
      mask Display: e = 0.06;c1 = [120 150 230]/255;c2 = ([120 150 230]+0)/383;c3 = ([120 150 230]+128)/383;patch([0 1 1 0],[0 0 1 1],c1);patch([0 1 1 1-e 1-e 0+e],[0 0 1 1-e 0+e 0+e],c2);patch([0 0 1 1-e 0+e 0+e],[0 1 1 1-e 1-e 0+e],c3);plot([0 1 1 0 0],[0 0 1 1 0]);disp('weights');
  "IW{2,1}(181,:)'" : Constant  Value=[1.702354944868516906097966057131998240947723388671875;1.413428640750062026398836678708903491497039794921875;-1.5200598817680883723113538508187048137187957763671875;-0.64109237728284440560599932723562233150005340576171875;-0.1404760264872709496497549253035685978829860687255859375;-1.56769637947871753880235701217316091060638427734375;-0.9809802030154728402777664086897857487201690673828125;-0.10495661618784056512421187790096155367791652679443359375]
      mask Display: e = 0.06;c1 = [120 150 230]/255;c2 = ([120 150 230]+0)/383;c3 = ([120 150 230]+128)/383;patch([0 1 1 0],[0 0 1 1],c1);patch([0 1 1 1-e 1-e 0+e],[0 0 1 1-e 0+e 0+e],c2);patch([0 0 1 1-e 0+e 0+e],[0 1 1 1-e 1-e 0+e],c3);plot([0 1 1 0 0],[0 0 1 1 0]);disp('weights');
  "IW{2,1}(182,:)'" : Constant  Value=[0.6790947557667477152421042774221859872341156005859375;-1.202245246031398817621038688230328261852264404296875;0.554323654715137337234409642405807971954345703125;1.2138767858814929478938893225858919322490692138671875;-1.0132414808655780813495539405266754329204559326171875;1.698217144304580816793759368010796606540679931640625;-1.702867995673071899176420629373751580715179443359375;0.668352774987109210513835932943038642406463623046875]
      mask Display: e = 0.06;c1 = [120 150 230]/255;c2 = ([120 150 230]+0)/383;c3 = ([120 150 230]+128)/383;patch([0 1 1 0],[0 0 1 1],c1);patch([0 1 1 1-e 1-e 0+e],[0 0 1 1-e 0+e 0+e],c2);patch([0 0 1 1-e 0+e 0+e],[0 1 1 1-e 1-e 0+e],c3);plot([0 1 1 0 0],[0 0 1 1 0]);disp('weights');
  "IW{2,1}(183,:)'" : Constant  Value=[2.05629124698634058177049155347049236297607421875;-1.01083198400857465770741328014992177486419677734375;-1.4071511077523675137257441747351549565792083740234375;-1.2504913164209898734924308882909826934337615966796875;0.022726305539532691557536026039088028483092784881591796875;0.51347379459376529808878331095911562442779541015625;1.1990894589594471852933565969578921794891357421875;-0.76349288670837134329616446848376654088497161865234375]
      mask Display: e = 0.06;c1 = [120 150 230]/255;c2 = ([120 150 230]+0)/383;c3 = ([120 150 230]+128)/383;patch([0 1 1 0],[0 0 1 1],c1);patch([0 1 1 1-e 1-e 0+e],[0 0 1 1-e 0+e 0+e],c2);patch([0 0 1 1-e 0+e 0+e],[0 1 1 1-e 1-e 0+e],c3);plot([0 1 1 0 0],[0 0 1 1 0]);disp('weights');
  "IW{2,1}(184,:)'" : Constant  Value=[0.7095272994476802264074422055273316800594329833984375;0.87998848462084444665975979660288430750370025634765625;-1.6414026655323772363459511325345374643802642822265625;0.63422889077218103093258605440496467053890228271484375;-0.84914118398189664116415542594040744006633758544921875;0.40866931323531174857777159559191204607486724853515625;1.3378343456902157537768971451441757380962371826171875;-1.97940200009672739867028212756849825382232666015625]
      mask Display: e = 0.06;c1 = [120 150 230]/255;c2 = ([120 150 230]+0)/383;c3 = ([120 150 230]+128)/383;patch([0 1 1 0],[0 0 1 1],c1);patch([0 1 1 1-e 1-e 0+e],[0 0 1 1-e 0+e 0+e],c2);patch([0 0 1 1-e 0+e 0+e],[0 1 1 1-e 1-e 0+e],c3);plot([0 1 1 0 0],[0 0 1 1 0]);disp('weights');
  "IW{2,1}(185,:)'" : Constant  Value=[-1.1277748920355377126867324477643705904483795166015625;0.46886281255551554014715520679601468145847320556640625;-1.930823709999963444516879462753422558307647705078125;-1.4561104859644069531299237496568821370601654052734375;-1.4585002980547268069955180180841125547885894775390625;0.803548147987018790416868796455673873424530029296875;-0.1317674914593090773617944932993850670754909515380859375;1.1890725218121165340789957554079592227935791015625]
      mask Display: e = 0.06;c1 = [120 150 230]/255;c2 = ([120 150 230]+0)/383;c3 = ([120 150 230]+128)/383;patch([0 1 1 0],[0 0 1 1],c1);patch([0 1 1 1-e 1-e 0+e],[0 0 1 1-e 0+e 0+e],c2);patch([0 0 1 1-e 0+e 0+e],[0 1 1 1-e 1-e 0+e],c3);plot([0 1 1 0 0],[0 0 1 1 0]);disp('weights');
  "IW{2,1}(186,:)'" : Constant  Value=[1.0259596740307894702226576555403880774974822998046875;-1.80423543345092785017413916648365557193756103515625;1.2426275675318765312482582885422743856906890869140625;-1.039547545804048400697183751617558300495147705078125;-1.0480905607410717639282893287600018084049224853515625;-0.1165945666977916683748617288074456155300140380859375;-1.43607750550254120724957829224877059459686279296875;-0.9581175653271518655174077139236032962799072265625]
      mask Display: e = 0.06;c1 = [120 150 230]/255;c2 = ([120 150 230]+0)/383;c3 = ([120 150 230]+128)/383;patch([0 1 1 0],[0 0 1 1],c1);patch([0 1 1 1-e 1-e 0+e],[0 0 1 1-e 0+e 0+e],c2);patch([0 0 1 1-e 0+e 0+e],[0 1 1 1-e 1-e 0+e],c3);plot([0 1 1 0 0],[0 0 1 1 0]);disp('weights');
  "IW{2,1}(187,:)'" : Constant  Value=[-0.73969505089516329743304368093959055840969085693359375;1.183388498350122386426619414123706519603729248046875;-1.6711759881870269506265458403504453599452972412109375;-0.945524969970393147633558328379876911640167236328125;0.71111970405177749032787914984510280191898345947265625;-0.476287092748067852898685714535531587898731231689453125;-1.744010386194349226940403241314925253391265869140625;-1.286380721108917324357889810926280915737152099609375]
      mask Display: e = 0.06;c1 = [120 150 230]/255;c2 = ([120 150 230]+0)/383;c3 = ([120 150 230]+128)/383;patch([0 1 1 0],[0 0 1 1],c1);patch([0 1 1 1-e 1-e 0+e],[0 0 1 1-e 0+e 0+e],c2);patch([0 0 1 1-e 0+e 0+e],[0 1 1 1-e 1-e 0+e],c3);plot([0 1 1 0 0],[0 0 1 1 0]);disp('weights');
  "IW{2,1}(188,:)'" : Constant  Value=[-0.2370386611768704465674773018690757453441619873046875;2.01313021189463370319572277367115020751953125;0.453827850659280940259776571110705845057964324951171875;-1.5755432379073639470590251221437938511371612548828125;0.0923462070810734114711948450349154882133007049560546875;-1.360747580540283774297449781442992389202117919921875;1.4671518471379056958170394864282570779323577880859375;0.462277806945601110744092920867842622101306915283203125]
      mask Display: e = 0.06;c1 = [120 150 230]/255;c2 = ([120 150 230]+0)/383;c3 = ([120 150 230]+128)/383;patch([0 1 1 0],[0 0 1 1],c1);patch([0 1 1 1-e 1-e 0+e],[0 0 1 1-e 0+e 0+e],c2);patch([0 0 1 1-e 0+e 0+e],[0 1 1 1-e 1-e 0+e],c3);plot([0 1 1 0 0],[0 0 1 1 0]);disp('weights');
  "IW{2,1}(189,:)'" : Constant  Value=[-1.6411528448342214137056771505740471184253692626953125;-0.73797741332577782014112699471297673881053924560546875;0.9126366107634040769625016764621250331401824951171875;1.0552868539607385134360129086417146027088165283203125;-1.5275278127844134079538207515724934637546539306640625;-0.657176243949245009190462951664812862873077392578125;-1.4866734986148084640689148727688007056713104248046875;0.99956779016834540474434334100806154310703277587890625]
      mask Display: e = 0.06;c1 = [120 150 230]/255;c2 = ([120 150 230]+0)/383;c3 = ([120 150 230]+128)/383;patch([0 1 1 0],[0 0 1 1],c1);patch([0 1 1 1-e 1-e 0+e],[0 0 1 1-e 0+e 0+e],c2);patch([0 0 1 1-e 0+e 0+e],[0 1 1 1-e 1-e 0+e],c3);plot([0 1 1 0 0],[0 0 1 1 0]);disp('weights');
  "IW{2,1}(19,:)'" : Constant  Value=[1.379612632176407505113502338645048439502716064453125;1.44984262305030764395041842362843453884124755859375;-0.3260121288336226275106355387833900749683380126953125;1.3659991162111275730950410434161312878131866455078125;1.46738008672590591885409594397060573101043701171875;-0.78513656357883843117662081567686982452869415283203125;1.133592380772023400226089506759308278560638427734375;1.0048194044249270096003101571113802492618560791015625]
      mask Display: e = 0.06;c1 = [120 150 230]/255;c2 = ([120 150 230]+0)/383;c3 = ([120 150 230]+128)/383;patch([0 1 1 0],[0 0 1 1],c1);patch([0 1 1 1-e 1-e 0+e],[0 0 1 1-e 0+e 0+e],c2);patch([0 0 1 1-e 0+e 0+e],[0 1 1 1-e 1-e 0+e],c3);plot([0 1 1 0 0],[0 0 1 1 0]);disp('weights');
  "IW{2,1}(190,:)'" : Constant  Value=[-0.272096970328696785568212135331123135983943939208984375;0.00556536418093342248603061506173617090098559856414794921875;1.826515632333338690074242549599148333072662353515625;-0.67844046373016742013106750164297409355640411376953125;1.6626401081554860184041899628937244415283203125;-1.9778615072899725646493607200682163238525390625;0.350835357390948399114449784974567592144012451171875;0.644405131304661704660929899546317756175994873046875]
      mask Display: e = 0.06;c1 = [120 150 230]/255;c2 = ([120 150 230]+0)/383;c3 = ([120 150 230]+128)/383;patch([0 1 1 0],[0 0 1 1],c1);patch([0 1 1 1-e 1-e 0+e],[0 0 1 1-e 0+e 0+e],c2);patch([0 0 1 1-e 0+e 0+e],[0 1 1 1-e 1-e 0+e],c3);plot([0 1 1 0 0],[0 0 1 1 0]);disp('weights');
  "IW{2,1}(191,:)'" : Constant  Value=[1.65095896190136404158010918763466179370880126953125;1.262956255419171558429525248357094824314117431640625;-1.7139769479154380871221974302898161113262176513671875;0.2965522838922025616881228415877558290958404541015625;0.471834738552097843200527904627961106598377227783203125;0.682099037736934032949420725344680249691009521484375;1.7543626637071636498177440444123931229114532470703125;0.182270759032965135038040216386434622108936309814453125]
      mask Display: e = 0.06;c1 = [120 150 230]/255;c2 = ([120 150 230]+0)/383;c3 = ([120 150 230]+128)/383;patch([0 1 1 0],[0 0 1 1],c1);patch([0 1 1 1-e 1-e 0+e],[0 0 1 1-e 0+e 0+e],c2);patch([0 0 1 1-e 0+e 0+e],[0 1 1 1-e 1-e 0+e],c3);plot([0 1 1 0 0],[0 0 1 1 0]);disp('weights');
  "IW{2,1}(192,:)'" : Constant  Value=[0.3920677954756637273447950065019540488719940185546875;-1.1014940197070435257131748585379682481288909912109375;1.4264731807798132212639075078186579048633575439453125;-0.71165975369703204922444683688809163868427276611328125;-0.2334626860689094918210884088694001547992229461669921875;-1.7807529241319144386324069273541681468486785888671875;1.120834954751212197976428797119297087192535400390625;-1.6306116608421741265289028888219036161899566650390625]
      mask Display: e = 0.06;c1 = [120 150 230]/255;c2 = ([120 150 230]+0)/383;c3 = ([120 150 230]+128)/383;patch([0 1 1 0],[0 0 1 1],c1);patch([0 1 1 1-e 1-e 0+e],[0 0 1 1-e 0+e 0+e],c2);patch([0 0 1 1-e 0+e 0+e],[0 1 1 1-e 1-e 0+e],c3);plot([0 1 1 0 0],[0 0 1 1 0]);disp('weights');
  "IW{2,1}(193,:)'" : Constant  Value=[1.67835181729590754429182197782211005687713623046875;0.570055054510981928928003981127403676509857177734375;1.9230076891827379004240583526552654802799224853515625;1.03642190687557889106074071605689823627471923828125;1.288149270434959081654824331053532660007476806640625;-0.45692213857701446944048484510858543217182159423828125;-0.8582202529329088225296118253027088940143585205078125;-0.428021645990926902225481853747623972594738006591796875]
      mask Display: e = 0.06;c1 = [120 150 230]/255;c2 = ([120 150 230]+0)/383;c3 = ([120 150 230]+128)/383;patch([0 1 1 0],[0 0 1 1],c1);patch([0 1 1 1-e 1-e 0+e],[0 0 1 1-e 0+e 0+e],c2);patch([0 0 1 1-e 0+e 0+e],[0 1 1 1-e 1-e 0+e],c3);plot([0 1 1 0 0],[0 0 1 1 0]);disp('weights');
  "IW{2,1}(194,:)'" : Constant  Value=[1.163547021369978562432834223727695643901824951171875;-0.7545784921053899640952522531733848154544830322265625;0.245959323338813262704860562735120765864849090576171875;-1.3286454567083521016712666096282191574573516845703125;1.179702292308492328487545819371007382869720458984375;-1.5568733489716433116001326197874732315540313720703125;1.3759322205506301362021304157678969204425811767578125;-1.2680434783519307639920725705451332032680511474609375]
      mask Display: e = 0.06;c1 = [120 150 230]/255;c2 = ([120 150 230]+0)/383;c3 = ([120 150 230]+128)/383;patch([0 1 1 0],[0 0 1 1],c1);patch([0 1 1 1-e 1-e 0+e],[0 0 1 1-e 0+e 0+e],c2);patch([0 0 1 1-e 0+e 0+e],[0 1 1 1-e 1-e 0+e],c3);plot([0 1 1 0 0],[0 0 1 1 0]);disp('weights');
  "IW{2,1}(195,:)'" : Constant  Value=[1.34842970517395865925891484948806464672088623046875;1.0244689879846002877883393011870793998241424560546875;-1.118790854448614258132010945701040327548980712890625;-1.476306506211225499924921678029932081699371337890625;-1.36676636803426987398779601790010929107666015625;0.73274140184313829582407606721972115337848663330078125;-1.2707304810902073644029997012694366276264190673828125;0.7391511224869014018423740708385594189167022705078125]
      mask Display: e = 0.06;c1 = [120 150 230]/255;c2 = ([120 150 230]+0)/383;c3 = ([120 150 230]+128)/383;patch([0 1 1 0],[0 0 1 1],c1);patch([0 1 1 1-e 1-e 0+e],[0 0 1 1-e 0+e 0+e],c2);patch([0 0 1 1-e 0+e 0+e],[0 1 1 1-e 1-e 0+e],c3);plot([0 1 1 0 0],[0 0 1 1 0]);disp('weights');
  "IW{2,1}(196,:)'" : Constant  Value=[0.55873240304268356748451651583309285342693328857421875;1.0287025693760176725533028729842044413089752197265625;1.574143104788076730216062060208059847354888916015625;-1.5397798144285863575220218990580178797245025634765625;-0.65765322509388746130554181945626623928546905517578125;-0.7206702225738883527128564310260117053985595703125;1.2462623092430689109022523552994243800640106201171875;-1.4164113753332572276377732123364694416522979736328125]
      mask Display: e = 0.06;c1 = [120 150 230]/255;c2 = ([120 150 230]+0)/383;c3 = ([120 150 230]+128)/383;patch([0 1 1 0],[0 0 1 1],c1);patch([0 1 1 1-e 1-e 0+e],[0 0 1 1-e 0+e 0+e],c2);patch([0 0 1 1-e 0+e 0+e],[0 1 1 1-e 1-e 0+e],c3);plot([0 1 1 0 0],[0 0 1 1 0]);disp('weights');
  "IW{2,1}(197,:)'" : Constant  Value=[1.5293203040920271273961361657711677253246307373046875;1.6518919817191155541280522811575792729854583740234375;0.90319948394150395554191845803870819509029388427734375;0.74833513327626588473862057071528397500514984130859375;0.1682458609393482074079173571590217761695384979248046875;1.2515892794456824343996004245127551257610321044921875;-1.2134219526817471290769390179775655269622802734375;-1.295197007329473404269037928315810859203338623046875]
      mask Display: e = 0.06;c1 = [120 150 230]/255;c2 = ([120 150 230]+0)/383;c3 = ([120 150 230]+128)/383;patch([0 1 1 0],[0 0 1 1],c1);patch([0 1 1 1-e 1-e 0+e],[0 0 1 1-e 0+e 0+e],c2);patch([0 0 1 1-e 0+e 0+e],[0 1 1 1-e 1-e 0+e],c3);plot([0 1 1 0 0],[0 0 1 1 0]);disp('weights');
  "IW{2,1}(198,:)'" : Constant  Value=[-1.891677011362522531356944455183111131191253662109375;1.6259739928468130987226913930498994886875152587890625;-0.59520466857242115832349327320116572082042694091796875;0.96010525250417544373959799486328847706317901611328125;-0.88112410317683675931021980431978590786457061767578125;0.011992048908752210578665398088560323230922222137451171875;1.6451568086425851777931939068366773426532745361328125;0.2408186001147644972331107737772981636226177215576171875]
      mask Display: e = 0.06;c1 = [120 150 230]/255;c2 = ([120 150 230]+0)/383;c3 = ([120 150 230]+128)/383;patch([0 1 1 0],[0 0 1 1],c1);patch([0 1 1 1-e 1-e 0+e],[0 0 1 1-e 0+e 0+e],c2);patch([0 0 1 1-e 0+e 0+e],[0 1 1 1-e 1-e 0+e],c3);plot([0 1 1 0 0],[0 0 1 1 0]);disp('weights');
  "IW{2,1}(199,:)'" : Constant  Value=[1.627792444831683393857701958040706813335418701171875;-1.8657692158841545637670833457377739250659942626953125;0.445100857935516291963295998357352800667285919189453125;1.3179455844675664888399069241131655871868133544921875;1.4072799028520481812165598967112600803375244140625;-0.69492598149459894329993403516709804534912109375;0.6164044332703884077062639335053972899913787841796875;0.72830245960566808438585439944290556013584136962890625]
      mask Display: e = 0.06;c1 = [120 150 230]/255;c2 = ([120 150 230]+0)/383;c3 = ([120 150 230]+128)/383;patch([0 1 1 0],[0 0 1 1],c1);patch([0 1 1 1-e 1-e 0+e],[0 0 1 1-e 0+e 0+e],c2);patch([0 0 1 1-e 0+e 0+e],[0 1 1 1-e 1-e 0+e],c3);plot([0 1 1 0 0],[0 0 1 1 0]);disp('weights');
  "IW{2,1}(2,:)'" : Constant  Value=[1.83637933881813264491711379378102719783782958984375;-1.2178066722543607891537931209313683211803436279296875;0.2600800620116652250857214312418363988399505615234375;-0.8622517449714910409142021308070980012416839599609375;0.330515502882989087307663567116833291947841644287109375;1.742346917420231289241883132490329444408416748046875;1.4585914335202077030118061884422786533832550048828125;-0.34382422113894450799165269927470944821834564208984375]
      mask Display: e = 0.06;c1 = [120 150 230]/255;c2 = ([120 150 230]+0)/383;c3 = ([120 150 230]+128)/383;patch([0 1 1 0],[0 0 1 1],c1);patch([0 1 1 1-e 1-e 0+e],[0 0 1 1-e 0+e 0+e],c2);patch([0 0 1 1-e 0+e 0+e],[0 1 1 1-e 1-e 0+e],c3);plot([0 1 1 0 0],[0 0 1 1 0]);disp('weights');
  "IW{2,1}(20,:)'" : Constant  Value=[-0.890652083995706167485195692279376089572906494140625;1.1800955864047910637282257084734737873077392578125;-1.9923586352904487650761211625649593770503997802734375;1.35829464494650142825094008003361523151397705078125;0.09115898025727771358805995305374381132423877716064453125;-0.288269836398222067952445968330721370875835418701171875;1.3226043000442888608603198008495382964611053466796875;-1.100427248050654061017894491669721901416778564453125]
      mask Display: e = 0.06;c1 = [120 150 230]/255;c2 = ([120 150 230]+0)/383;c3 = ([120 150 230]+128)/383;patch([0 1 1 0],[0 0 1 1],c1);patch([0 1 1 1-e 1-e 0+e],[0 0 1 1-e 0+e 0+e],c2);patch([0 0 1 1-e 0+e 0+e],[0 1 1 1-e 1-e 0+e],c3);plot([0 1 1 0 0],[0 0 1 1 0]);disp('weights');
  "IW{2,1}(200,:)'" : Constant  Value=[-0.72806924019865615349544896162115037441253662109375;0.5623555475715023010963022898067720234394073486328125;-1.6372705956566486751313505010330118238925933837890625;-1.0033686115159528018381251968094147741794586181640625;-1.4851939755721257352405473284306935966014862060546875;1.949275225194942340323223106679506599903106689453125;0.15754662808399422235794418156729079782962799072265625;0.6716864400628177467211799012147821485996246337890625]
      mask Display: e = 0.06;c1 = [120 150 230]/255;c2 = ([120 150 230]+0)/383;c3 = ([120 150 230]+128)/383;patch([0 1 1 0],[0 0 1 1],c1);patch([0 1 1 1-e 1-e 0+e],[0 0 1 1-e 0+e 0+e],c2);patch([0 0 1 1-e 0+e 0+e],[0 1 1 1-e 1-e 0+e],c3);plot([0 1 1 0 0],[0 0 1 1 0]);disp('weights');
  "IW{2,1}(201,:)'" : Constant  Value=[1.7575907808407624788316070407745428383350372314453125;-1.853106296974822431167240210925228893756866455078125;-0.739240667436606546658595107146538794040679931640625;-1.43098085470740787883414668613113462924957275390625;-0.09114178358922142564324531122110784053802490234375;0.652644970043322114605643946561031043529510498046875;1.1814235323203992056306788072106428444385528564453125;0.43778342983326468118576713095535524189472198486328125]
      mask Display: e = 0.06;c1 = [120 150 230]/255;c2 = ([120 150 230]+0)/383;c3 = ([120 150 230]+128)/383;patch([0 1 1 0],[0 0 1 1],c1);patch([0 1 1 1-e 1-e 0+e],[0 0 1 1-e 0+e 0+e],c2);patch([0 0 1 1-e 0+e 0+e],[0 1 1 1-e 1-e 0+e],c3);plot([0 1 1 0 0],[0 0 1 1 0]);disp('weights');
  "IW{2,1}(202,:)'" : Constant  Value=[1.5527173682896970863254182404489256441593170166015625;-1.0948273399139563100135319473338313400745391845703125;1.0814492686169170365673153355601243674755096435546875;-0.403437382437156266679068039593403227627277374267578125;1.4039142694930861754443185418494977056980133056640625;-1.756370480502996489491351894685067236423492431640625;0.94251327076925883741154166273190639913082122802734375;-0.381351313262794533454069778599659912288188934326171875]
      mask Display: e = 0.06;c1 = [120 150 230]/255;c2 = ([120 150 230]+0)/383;c3 = ([120 150 230]+128)/383;patch([0 1 1 0],[0 0 1 1],c1);patch([0 1 1 1-e 1-e 0+e],[0 0 1 1-e 0+e 0+e],c2);patch([0 0 1 1-e 0+e 0+e],[0 1 1 1-e 1-e 0+e],c3);plot([0 1 1 0 0],[0 0 1 1 0]);disp('weights');
  "IW{2,1}(203,:)'" : Constant  Value=[-0.309170633181494236563224831115803681313991546630859375;-0.662814005248665960579046441125683486461639404296875;1.5473068968061358674503935617394745349884033203125;1.8100260742858600426785642412141896784305572509765625;0.9596251569455287455667757967603392899036407470703125;-1.1091246979373268199964286395697854459285736083984375;0.41061463205197679116054132464341819286346435546875;1.5777791482730183503235821262933313846588134765625]
      mask Display: e = 0.06;c1 = [120 150 230]/255;c2 = ([120 150 230]+0)/383;c3 = ([120 150 230]+128)/383;patch([0 1 1 0],[0 0 1 1],c1);patch([0 1 1 1-e 1-e 0+e],[0 0 1 1-e 0+e 0+e],c2);patch([0 0 1 1-e 0+e 0+e],[0 1 1 1-e 1-e 0+e],c3);plot([0 1 1 0 0],[0 0 1 1 0]);disp('weights');
  "IW{2,1}(204,:)'" : Constant  Value=[1.34672043031116839273408913868479430675506591796875;1.6022759779221822373784789306228049099445343017578125;0.979783008642480357508475208305753767490386962890625;-0.789666987225305927466934008407406508922576904296875;1.6832159811400642102086067097843624651432037353515625;-0.96212678004927543184976457268930971622467041015625;-0.1509116942860524723801773916420643217861652374267578125;1.0685052834615758055036849327734671533107757568359375]
      mask Display: e = 0.06;c1 = [120 150 230]/255;c2 = ([120 150 230]+0)/383;c3 = ([120 150 230]+128)/383;patch([0 1 1 0],[0 0 1 1],c1);patch([0 1 1 1-e 1-e 0+e],[0 0 1 1-e 0+e 0+e],c2);patch([0 0 1 1-e 0+e 0+e],[0 1 1 1-e 1-e 0+e],c3);plot([0 1 1 0 0],[0 0 1 1 0]);disp('weights');
  "IW{2,1}(205,:)'" : Constant  Value=[1.45023657196794264478967306786216795444488525390625;0.031196945790084425198518403021807898767292499542236328125;0.70772348182609856603875186920049600303173065185546875;1.451725730377035450402445349027402698993682861328125;-1.6250230739796014400866397409117780625820159912109375;-0.1933035716554080962747974581361631862819194793701171875;0.5325714920111987993323054979555308818817138671875;-1.82308252968614947775449763867072761058807373046875]
      mask Display: e = 0.06;c1 = [120 150 230]/255;c2 = ([120 150 230]+0)/383;c3 = ([120 150 230]+128)/383;patch([0 1 1 0],[0 0 1 1],c1);patch([0 1 1 1-e 1-e 0+e],[0 0 1 1-e 0+e 0+e],c2);patch([0 0 1 1-e 0+e 0+e],[0 1 1 1-e 1-e 0+e],c3);plot([0 1 1 0 0],[0 0 1 1 0]);disp('weights');
  "IW{2,1}(206,:)'" : Constant  Value=[-1.563825662985661946180471204570494592189788818359375;-0.9175372397190086903862038525403477251529693603515625;1.256619701194665150723039914737455546855926513671875;-2.048251548997502169413564843125641345977783203125;0.455783749927485770658819319578469730913639068603515625;0.97450134961508438902200168740819208323955535888671875;-0.757020992021234295776821454637683928012847900390625;0.493512471999732083016709793810150586068630218505859375]
      mask Display: e = 0.06;c1 = [120 150 230]/255;c2 = ([120 150 230]+0)/383;c3 = ([120 150 230]+128)/383;patch([0 1 1 0],[0 0 1 1],c1);patch([0 1 1 1-e 1-e 0+e],[0 0 1 1-e 0+e 0+e],c2);patch([0 0 1 1-e 0+e 0+e],[0 1 1 1-e 1-e 0+e],c3);plot([0 1 1 0 0],[0 0 1 1 0]);disp('weights');
  "IW{2,1}(207,:)'" : Constant  Value=[0.0960025133301881938852062603473314084112644195556640625;-1.442826230702589640486621647141873836517333984375;-0.68532216917608501649539221034501679241657257080078125;-1.8903000002227419162892374515649862587451934814453125;1.43233578829587759884134356980212032794952392578125;-1.1380283632611725153083170880563557147979736328125;-1.0608770153671323033250928347115404903888702392578125;-0.65584159532209940213220988880493678152561187744140625]
      mask Display: e = 0.06;c1 = [120 150 230]/255;c2 = ([120 150 230]+0)/383;c3 = ([120 150 230]+128)/383;patch([0 1 1 0],[0 0 1 1],c1);patch([0 1 1 1-e 1-e 0+e],[0 0 1 1-e 0+e 0+e],c2);patch([0 0 1 1-e 0+e 0+e],[0 1 1 1-e 1-e 0+e],c3);plot([0 1 1 0 0],[0 0 1 1 0]);disp('weights');
  "IW{2,1}(208,:)'" : Constant  Value=[1.48535186281059328194942281697876751422882080078125;-0.1753032612959353198078815694316290318965911865234375;-1.506626351416330056309789142687804996967315673828125;0.80482416007397084012353616344626061618328094482421875;-0.3189667354556473544135997144621796905994415283203125;1.6487366040485589291364476594026200473308563232421875;-1.5267285458035628753492574105621315538883209228515625;-0.82558972900029814478983780645648948848247528076171875]
      mask Display: e = 0.06;c1 = [120 150 230]/255;c2 = ([120 150 230]+0)/383;c3 = ([120 150 230]+128)/383;patch([0 1 1 0],[0 0 1 1],c1);patch([0 1 1 1-e 1-e 0+e],[0 0 1 1-e 0+e 0+e],c2);patch([0 0 1 1-e 0+e 0+e],[0 1 1 1-e 1-e 0+e],c3);plot([0 1 1 0 0],[0 0 1 1 0]);disp('weights');
  "IW{2,1}(209,:)'" : Constant  Value=[-0.0289847098599668347163049730852435459382832050323486328125;-0.2447283725748331251192979607367306016385555267333984375;1.4675121682650520416046902028028853237628936767578125;1.5735714586872686648888475247076712548732757568359375;1.3692484431149265500238243475905619561672210693359375;-1.1354577351202801427376698484295047819614410400390625;1.548920746667084014092097277170978486537933349609375;-0.87893553310931971100927739826147444546222686767578125]
      mask Display: e = 0.06;c1 = [120 150 230]/255;c2 = ([120 150 230]+0)/383;c3 = ([120 150 230]+128)/383;patch([0 1 1 0],[0 0 1 1],c1);patch([0 1 1 1-e 1-e 0+e],[0 0 1 1-e 0+e 0+e],c2);patch([0 0 1 1-e 0+e 0+e],[0 1 1 1-e 1-e 0+e],c3);plot([0 1 1 0 0],[0 0 1 1 0]);disp('weights');
  "IW{2,1}(21,:)'" : Constant  Value=[-1.139237912389526652390259187086485326290130615234375;0.79853720880777245838544331490993499755859375;0.88802507928903595679770432980149053037166595458984375;1.340949900503350722402728933957405388355255126953125;0.95500021744171259552302899464848451316356658935546875;-1.4002596191368017475298302088049240410327911376953125;0.24146100701048478498478289111517369747161865234375;1.8881125941933791789750785028445534408092498779296875]
      mask Display: e = 0.06;c1 = [120 150 230]/255;c2 = ([120 150 230]+0)/383;c3 = ([120 150 230]+128)/383;patch([0 1 1 0],[0 0 1 1],c1);patch([0 1 1 1-e 1-e 0+e],[0 0 1 1-e 0+e 0+e],c2);patch([0 0 1 1-e 0+e 0+e],[0 1 1 1-e 1-e 0+e],c3);plot([0 1 1 0 0],[0 0 1 1 0]);disp('weights');
  "IW{2,1}(210,:)'" : Constant  Value=[-1.4550570882428246477502398192882537841796875;-1.3919105200312469339252174904686398804187774658203125;-0.1377313135349752803993084171452210284769535064697265625;-1.501269706639255741009719713474623858928680419921875;-0.77200462164890193417221553318086080253124237060546875;1.565801287432768251761672217980958521366119384765625;-0.10726933809123850860345328328548930585384368896484375;-1.2797746414214794530295193908386863768100738525390625]
      mask Display: e = 0.06;c1 = [120 150 230]/255;c2 = ([120 150 230]+0)/383;c3 = ([120 150 230]+128)/383;patch([0 1 1 0],[0 0 1 1],c1);patch([0 1 1 1-e 1-e 0+e],[0 0 1 1-e 0+e 0+e],c2);patch([0 0 1 1-e 0+e 0+e],[0 1 1 1-e 1-e 0+e],c3);plot([0 1 1 0 0],[0 0 1 1 0]);disp('weights');
  "IW{2,1}(211,:)'" : Constant  Value=[0.577116449947208121074027076247148215770721435546875;-0.7239907928984614660095076033030636608600616455078125;1.881284333047850143572077286080457270145416259765625;-1.32885573031669945720523173804394900798797607421875;-1.3410059900107580421746433785301633179187774658203125;0.63103885593417874400046230221050791442394256591796875;-1.54316928946604381422957885661162436008453369140625;0.5369213955582774477903740262263454496860504150390625]
      mask Display: e = 0.06;c1 = [120 150 230]/255;c2 = ([120 150 230]+0)/383;c3 = ([120 150 230]+128)/383;patch([0 1 1 0],[0 0 1 1],c1);patch([0 1 1 1-e 1-e 0+e],[0 0 1 1-e 0+e 0+e],c2);patch([0 0 1 1-e 0+e 0+e],[0 1 1 1-e 1-e 0+e],c3);plot([0 1 1 0 0],[0 0 1 1 0]);disp('weights');
  "IW{2,1}(212,:)'" : Constant  Value=[-0.83915267470162568930192037441884167492389678955078125;-1.8399243364605479822415645685396157205104827880859375;-1.6505266923168055992476865867502056062221527099609375;1.3964283229394875984752388831111602485179901123046875;-0.413497477779297850641881950650713406503200531005859375;-0.7225844135725696393279804397025145590305328369140625;-0.3974810229669920591533127662842161953449249267578125;-1.2506130615403499017901367551530711352825164794921875]
      mask Display: e = 0.06;c1 = [120 150 230]/255;c2 = ([120 150 230]+0)/383;c3 = ([120 150 230]+128)/383;patch([0 1 1 0],[0 0 1 1],c1);patch([0 1 1 1-e 1-e 0+e],[0 0 1 1-e 0+e 0+e],c2);patch([0 0 1 1-e 0+e 0+e],[0 1 1 1-e 1-e 0+e],c3);plot([0 1 1 0 0],[0 0 1 1 0]);disp('weights');
  "IW{2,1}(213,:)'" : Constant  Value=[0.06370977945872613457112265678006224334239959716796875;-1.1967321266641792743001815324532799422740936279296875;0.061530859310181977572806744092304143123328685760498046875;1.6864368812123802232605385142960585653781890869140625;-1.7762074764486250888495533217792399227619171142578125;-0.485019621181350724103964466848992742598056793212890625;-0.5318696850511710483289107287419028580188751220703125;-1.7483596629458395543821325190947391092777252197265625]
      mask Display: e = 0.06;c1 = [120 150 230]/255;c2 = ([120 150 230]+0)/383;c3 = ([120 150 230]+128)/383;patch([0 1 1 0],[0 0 1 1],c1);patch([0 1 1 1-e 1-e 0+e],[0 0 1 1-e 0+e 0+e],c2);patch([0 0 1 1-e 0+e 0+e],[0 1 1 1-e 1-e 0+e],c3);plot([0 1 1 0 0],[0 0 1 1 0]);disp('weights');
  "IW{2,1}(214,:)'" : Constant  Value=[-1.33223009029337102759882327518425881862640380859375;0.44695981487425717748607212342903949320316314697265625;2.081939898443845304853994093718938529491424560546875;-0.723702112144401166204943365301005542278289794921875;-1.7669070545876655042860647881752811372280120849609375;0.7005602060863207469765256973914802074432373046875;-0.8647069823412778521998234282364137470722198486328125;-0.21830268296948973638649249551235698163509368896484375]
      mask Display: e = 0.06;c1 = [120 150 230]/255;c2 = ([120 150 230]+0)/383;c3 = ([120 150 230]+128)/383;patch([0 1 1 0],[0 0 1 1],c1);patch([0 1 1 1-e 1-e 0+e],[0 0 1 1-e 0+e 0+e],c2);patch([0 0 1 1-e 0+e 0+e],[0 1 1 1-e 1-e 0+e],c3);plot([0 1 1 0 0],[0 0 1 1 0]);disp('weights');
  "IW{2,1}(215,:)'" : Constant  Value=[-0.5376540384719652454492688775644637644290924072265625;-0.668309572905391835462296512559987604618072509765625;-0.9599894483470354789034217901644296944141387939453125;-2.2510696388438731219139299355447292327880859375;1.21778604670581902524872930371202528476715087890625;-1.2903768920610054760089724368299357593059539794921875;-0.353507554043061944515358163698692806065082550048828125;-1.104970342551753414994664126425050199031829833984375]
      mask Display: e = 0.06;c1 = [120 150 230]/255;c2 = ([120 150 230]+0)/383;c3 = ([120 150 230]+128)/383;patch([0 1 1 0],[0 0 1 1],c1);patch([0 1 1 1-e 1-e 0+e],[0 0 1 1-e 0+e 0+e],c2);patch([0 0 1 1-e 0+e 0+e],[0 1 1 1-e 1-e 0+e],c3);plot([0 1 1 0 0],[0 0 1 1 0]);disp('weights');
  "IW{2,1}(216,:)'" : Constant  Value=[-2.211483395565294163276348626823164522647857666015625;0.5695078383816551959029084173380397260189056396484375;1.494752247198326333688100930885411798954010009765625;-1.01530401060654451583786794799380004405975341796875;-0.61213479965991102194067252639797516167163848876953125;-0.097179052355497341775247832629247568547725677490234375;1.5591944097132988122922370166634209454059600830078125;-0.1457544822382228488777400343678891658782958984375]
      mask Display: e = 0.06;c1 = [120 150 230]/255;c2 = ([120 150 230]+0)/383;c3 = ([120 150 230]+128)/383;patch([0 1 1 0],[0 0 1 1],c1);patch([0 1 1 1-e 1-e 0+e],[0 0 1 1-e 0+e 0+e],c2);patch([0 0 1 1-e 0+e 0+e],[0 1 1 1-e 1-e 0+e],c3);plot([0 1 1 0 0],[0 0 1 1 0]);disp('weights');
  "IW{2,1}(217,:)'" : Constant  Value=[-1.64764956407757257039747855742461979389190673828125;1.4443817905655091937688894176972098648548126220703125;0.9222620468091913270569648375385440886020660400390625;0.18799698193644187593775995992473326623439788818359375;-1.0394802135730938363877839947235770523548126220703125;-0.9735765940510372473681854899041354656219482421875;0.0560498933040605440414339000199106521904468536376953125;-1.796700699182775640139198003453202545642852783203125]
      mask Display: e = 0.06;c1 = [120 150 230]/255;c2 = ([120 150 230]+0)/383;c3 = ([120 150 230]+128)/383;patch([0 1 1 0],[0 0 1 1],c1);patch([0 1 1 1-e 1-e 0+e],[0 0 1 1-e 0+e 0+e],c2);patch([0 0 1 1-e 0+e 0+e],[0 1 1 1-e 1-e 0+e],c3);plot([0 1 1 0 0],[0 0 1 1 0]);disp('weights');
  "IW{2,1}(218,:)'" : Constant  Value=[0.46686101783750777460824110676185227930545806884765625;1.8986499005945274287654456202290020883083343505859375;-0.491288573829816666016512272108229808509349822998046875;-0.58366147490995345936681815146584995090961456298828125;0.78680400599122479743385838446556590497493743896484375;-1.4544775472290469853220429286011494696140289306640625;1.5627734604667191664617575952433981001377105712890625;1.1747426908456584104811781799071468412876129150390625]
      mask Display: e = 0.06;c1 = [120 150 230]/255;c2 = ([120 150 230]+0)/383;c3 = ([120 150 230]+128)/383;patch([0 1 1 0],[0 0 1 1],c1);patch([0 1 1 1-e 1-e 0+e],[0 0 1 1-e 0+e 0+e],c2);patch([0 0 1 1-e 0+e 0+e],[0 1 1 1-e 1-e 0+e],c3);plot([0 1 1 0 0],[0 0 1 1 0]);disp('weights');
  "IW{2,1}(219,:)'" : Constant  Value=[-1.089922087242005677154566001263447105884552001953125;1.551967690696964385921319262706674635410308837890625;-1.83759474306495551587659065262414515018463134765625;0.3365062544264201260801883108797483146190643310546875;-0.38056857022328161033186688655405305325984954833984375;-0.11028473362431649718029547102560172788798809051513671875;1.5612130488202911049455678949016146361827850341796875;1.145326230135438105861567237298004329204559326171875]
      mask Display: e = 0.06;c1 = [120 150 230]/255;c2 = ([120 150 230]+0)/383;c3 = ([120 150 230]+128)/383;patch([0 1 1 0],[0 0 1 1],c1);patch([0 1 1 1-e 1-e 0+e],[0 0 1 1-e 0+e 0+e],c2);patch([0 0 1 1-e 0+e 0+e],[0 1 1 1-e 1-e 0+e],c3);plot([0 1 1 0 0],[0 0 1 1 0]);disp('weights');
  "IW{2,1}(22,:)'" : Constant  Value=[-0.423314741043494147110237690867506898939609527587890625;-1.0997334003561067827803299223887734115123748779296875;-1.30491392732261513032199218287132680416107177734375;-0.94068805225923102231178063448169268667697906494140625;-1.1827387560827606893809615939971990883350372314453125;1.416511759893044342106804833747446537017822265625;1.246426958475019386440862945164553821086883544921875;1.2728125888523507125427158825914375483989715576171875]
      mask Display: e = 0.06;c1 = [120 150 230]/255;c2 = ([120 150 230]+0)/383;c3 = ([120 150 230]+128)/383;patch([0 1 1 0],[0 0 1 1],c1);patch([0 1 1 1-e 1-e 0+e],[0 0 1 1-e 0+e 0+e],c2);patch([0 0 1 1-e 0+e 0+e],[0 1 1 1-e 1-e 0+e],c3);plot([0 1 1 0 0],[0 0 1 1 0]);disp('weights');
  "IW{2,1}(220,:)'" : Constant  Value=[-0.1459345119969937820680883078239276073873043060302734375;-0.93486790791046969761879381621838547289371490478515625;1.1580099534365853042316985010984353721141815185546875;0.383104002094182105597752752146334387362003326416015625;0.80655935552157542733908712762058712542057037353515625;1.6687946017922306030101253782049752771854400634765625;2.1204905217452303389791268273256719112396240234375;0.83996022594845276554309521088725887238979339599609375]
      mask Display: e = 0.06;c1 = [120 150 230]/255;c2 = ([120 150 230]+0)/383;c3 = ([120 150 230]+128)/383;patch([0 1 1 0],[0 0 1 1],c1);patch([0 1 1 1-e 1-e 0+e],[0 0 1 1-e 0+e 0+e],c2);patch([0 0 1 1-e 0+e 0+e],[0 1 1 1-e 1-e 0+e],c3);plot([0 1 1 0 0],[0 0 1 1 0]);disp('weights');
  "IW{2,1}(221,:)'" : Constant  Value=[-0.10597658696631118147024608333595097064971923828125;0.2140206907535626978944520715231192298233509063720703125;-0.56909365862336380725849949158146046102046966552734375;-1.5347918246133074315906696938327513635158538818359375;0.83257167642571772159243437272380106151103973388671875;2.57456094800564283531230103108100593090057373046875;-0.96833992610767605224708631794783286750316619873046875;0.260938909475784852620705578374327160418033599853515625]
      mask Display: e = 0.06;c1 = [120 150 230]/255;c2 = ([120 150 230]+0)/383;c3 = ([120 150 230]+128)/383;patch([0 1 1 0],[0 0 1 1],c1);patch([0 1 1 1-e 1-e 0+e],[0 0 1 1-e 0+e 0+e],c2);patch([0 0 1 1-e 0+e 0+e],[0 1 1 1-e 1-e 0+e],c3);plot([0 1 1 0 0],[0 0 1 1 0]);disp('weights');
  "IW{2,1}(222,:)'" : Constant  Value=[1.6647468047925839673695236342609860002994537353515625;-0.269334601256818906289680626287008635699748992919921875;-1.4933101530609997897869334337883628904819488525390625;-0.7871388211529894984863631179905496537685394287109375;1.449427658826806464276160113513469696044921875;-1.3077755764629428458789561773301102221012115478515625;1.2241622096894519966525649579125456511974334716796875;0.016824148488373401322260036749867140315473079681396484375]
      mask Display: e = 0.06;c1 = [120 150 230]/255;c2 = ([120 150 230]+0)/383;c3 = ([120 150 230]+128)/383;patch([0 1 1 0],[0 0 1 1],c1);patch([0 1 1 1-e 1-e 0+e],[0 0 1 1-e 0+e 0+e],c2);patch([0 0 1 1-e 0+e 0+e],[0 1 1 1-e 1-e 0+e],c3);plot([0 1 1 0 0],[0 0 1 1 0]);disp('weights');
  "IW{2,1}(223,:)'" : Constant  Value=[1.9355959343341047063091764357523061335086822509765625;0.38867289264510507251770832226611673831939697265625;0.87207778738251906514022948613273911178112030029296875;-0.9635922338783402540940414837677963078022003173828125;-0.67495142221511994495841690877568908035755157470703125;-0.8870907835303736277410280308686196804046630859375;-1.066105657771922121668239924474619328975677490234375;-1.7831094333107484484202132080099545419216156005859375]
      mask Display: e = 0.06;c1 = [120 150 230]/255;c2 = ([120 150 230]+0)/383;c3 = ([120 150 230]+128)/383;patch([0 1 1 0],[0 0 1 1],c1);patch([0 1 1 1-e 1-e 0+e],[0 0 1 1-e 0+e 0+e],c2);patch([0 0 1 1-e 0+e 0+e],[0 1 1 1-e 1-e 0+e],c3);plot([0 1 1 0 0],[0 0 1 1 0]);disp('weights');
  "IW{2,1}(224,:)'" : Constant  Value=[-0.205995691832049521163838790016598068177700042724609375;-1.3956066319848334789099908448406495153903961181640625;1.562562321727252179215383875998668372631072998046875;-0.2403524996844164096643226002925075590610504150390625;-1.3515632960005723450791492723510600626468658447265625;0.7693446662014353787384379756986163556575775146484375;1.28002622441297564392925778520293533802032470703125;1.59479856228461702727372539811767637729644775390625]
      mask Display: e = 0.06;c1 = [120 150 230]/255;c2 = ([120 150 230]+0)/383;c3 = ([120 150 230]+128)/383;patch([0 1 1 0],[0 0 1 1],c1);patch([0 1 1 1-e 1-e 0+e],[0 0 1 1-e 0+e 0+e],c2);patch([0 0 1 1-e 0+e 0+e],[0 1 1 1-e 1-e 0+e],c3);plot([0 1 1 0 0],[0 0 1 1 0]);disp('weights');
  "IW{2,1}(225,:)'" : Constant  Value=[1.457276766447967109030514620826579630374908447265625;0.22581432019729452687073489869362674653530120849609375;-0.5158338635361496837816730476333759725093841552734375;2.4023219368882937629905427456833422183990478515625;0.0229117505118495608240625216467378777451813220977783203125;-0.872694307131692159629210436833091080188751220703125;0.0813392790598047865646691434449166990816593170166015625;-1.424931556724696957161313548567704856395721435546875]
      mask Display: e = 0.06;c1 = [120 150 230]/255;c2 = ([120 150 230]+0)/383;c3 = ([120 150 230]+128)/383;patch([0 1 1 0],[0 0 1 1],c1);patch([0 1 1 1-e 1-e 0+e],[0 0 1 1-e 0+e 0+e],c2);patch([0 0 1 1-e 0+e 0+e],[0 1 1 1-e 1-e 0+e],c3);plot([0 1 1 0 0],[0 0 1 1 0]);disp('weights');
  "IW{2,1}(226,:)'" : Constant  Value=[-0.66473668737727320543484665904543362557888031005859375;-1.971862813607004216720497424830682575702667236328125;-2.212305107598416586967005059705115854740142822265625;-0.397985893293952841531790909357368946075439453125;-0.747458365267778646057195146568119525909423828125;-0.5081704001250371138809214244247414171695709228515625;-0.472676320594250742868069892210769467055797576904296875;-0.80433758108456654412066200166009366512298583984375]
      mask Display: e = 0.06;c1 = [120 150 230]/255;c2 = ([120 150 230]+0)/383;c3 = ([120 150 230]+128)/383;patch([0 1 1 0],[0 0 1 1],c1);patch([0 1 1 1-e 1-e 0+e],[0 0 1 1-e 0+e 0+e],c2);patch([0 0 1 1-e 0+e 0+e],[0 1 1 1-e 1-e 0+e],c3);plot([0 1 1 0 0],[0 0 1 1 0]);disp('weights');
  "IW{2,1}(227,:)'" : Constant  Value=[-1.8321020488646426738199579631327651441097259521484375;0.7652539204931902983020108877099119126796722412109375;-0.7581970101290809171956652789958752691745758056640625;-1.6934302193639465539121147230616770684719085693359375;-0.99279535414916553204278670818894170224666595458984375;-1.510740726484647300509323031292296946048736572265625;0.72146909166921691092255741750705055892467498779296875;0.378176232568631587316332343107205815613269805908203125]
      mask Display: e = 0.06;c1 = [120 150 230]/255;c2 = ([120 150 230]+0)/383;c3 = ([120 150 230]+128)/383;patch([0 1 1 0],[0 0 1 1],c1);patch([0 1 1 1-e 1-e 0+e],[0 0 1 1-e 0+e 0+e],c2);patch([0 0 1 1-e 0+e 0+e],[0 1 1 1-e 1-e 0+e],c3);plot([0 1 1 0 0],[0 0 1 1 0]);disp('weights');
  "IW{2,1}(228,:)'" : Constant  Value=[-1.229412826439205463913140192744322121143341064453125;-0.650956521688341727127635749639011919498443603515625;-1.493518170830727687103944845148362219333648681640625;0.89328576869237708013571364062954671680927276611328125;-0.36931466697955672717768038637586869299411773681640625;1.982273397269393999664544026018120348453521728515625;-0.9939382119422963679511440204805694520473480224609375;-0.85499334002513072139350924771861173212528228759765625]
      mask Display: e = 0.06;c1 = [120 150 230]/255;c2 = ([120 150 230]+0)/383;c3 = ([120 150 230]+128)/383;patch([0 1 1 0],[0 0 1 1],c1);patch([0 1 1 1-e 1-e 0+e],[0 0 1 1-e 0+e 0+e],c2);patch([0 0 1 1-e 0+e 0+e],[0 1 1 1-e 1-e 0+e],c3);plot([0 1 1 0 0],[0 0 1 1 0]);disp('weights');
  "IW{2,1}(229,:)'" : Constant  Value=[1.8251574375981334252827537056873552501201629638671875;-0.62153305614150300417719563483842648565769195556640625;1.8887125519115126603963972229394130408763885498046875;-1.2357672115292503978167815148481167852878570556640625;1.1472446680675620900302646987256594002246856689453125;0.84481808151496551317904959432780742645263671875;-0.119116406613110348278183892034576274454593658447265625;0.6430509895073697190781558674643747508525848388671875]
      mask Display: e = 0.06;c1 = [120 150 230]/255;c2 = ([120 150 230]+0)/383;c3 = ([120 150 230]+128)/383;patch([0 1 1 0],[0 0 1 1],c1);patch([0 1 1 1-e 1-e 0+e],[0 0 1 1-e 0+e 0+e],c2);patch([0 0 1 1-e 0+e 0+e],[0 1 1 1-e 1-e 0+e],c3);plot([0 1 1 0 0],[0 0 1 1 0]);disp('weights');
  "IW{2,1}(23,:)'" : Constant  Value=[1.2343137503887289252446635146043263375759124755859375;2.2150563895450137152920433436520397663116455078125;0.374736731454777538541378589798114262521266937255859375;0.72199567020990629284682427169173024594783782958984375;0.8652674239956168467102770591736771166324615478515625;1.337473587481016412681356086977757513523101806640625;0.12541086087120045799991885360213927924633026123046875;-1.1570988951642362518867912513087503612041473388671875]
      mask Display: e = 0.06;c1 = [120 150 230]/255;c2 = ([120 150 230]+0)/383;c3 = ([120 150 230]+128)/383;patch([0 1 1 0],[0 0 1 1],c1);patch([0 1 1 1-e 1-e 0+e],[0 0 1 1-e 0+e 0+e],c2);patch([0 0 1 1-e 0+e 0+e],[0 1 1 1-e 1-e 0+e],c3);plot([0 1 1 0 0],[0 0 1 1 0]);disp('weights');
  "IW{2,1}(230,:)'" : Constant  Value=[-1.9721056451857263969174027806730009615421295166015625;0.77884578701228790453825467920978553593158721923828125;0.150944346450618771537932616411126218736171722412109375;0.87849303146057133862001364832394756376743316650390625;1.59452731155184768141452877898700535297393798828125;-0.33969889098091254897582302874070592224597930908203125;0.62853723914255021920638455412699840962886810302734375;-1.6244471320281650417172158995526842772960662841796875]
      mask Display: e = 0.06;c1 = [120 150 230]/255;c2 = ([120 150 230]+0)/383;c3 = ([120 150 230]+128)/383;patch([0 1 1 0],[0 0 1 1],c1);patch([0 1 1 1-e 1-e 0+e],[0 0 1 1-e 0+e 0+e],c2);patch([0 0 1 1-e 0+e 0+e],[0 1 1 1-e 1-e 0+e],c3);plot([0 1 1 0 0],[0 0 1 1 0]);disp('weights');
  "IW{2,1}(231,:)'" : Constant  Value=[-1.6355547552180069725835664939950220286846160888671875;-0.004204767138426651097715680549526950926519930362701416015625;-1.5313939562651619485933451869641430675983428955078125;1.504491591856602639154516509734094142913818359375;-0.6665584948941483123263651577872224152088165283203125;-0.92276733968372237626454079872928559780120849609375;1.5665598169561329999766030596219934523105621337890625;0.47385709054276947682637910475023090839385986328125]
      mask Display: e = 0.06;c1 = [120 150 230]/255;c2 = ([120 150 230]+0)/383;c3 = ([120 150 230]+128)/383;patch([0 1 1 0],[0 0 1 1],c1);patch([0 1 1 1-e 1-e 0+e],[0 0 1 1-e 0+e 0+e],c2);patch([0 0 1 1-e 0+e 0+e],[0 1 1 1-e 1-e 0+e],c3);plot([0 1 1 0 0],[0 0 1 1 0]);disp('weights');
  "IW{2,1}(232,:)'" : Constant  Value=[-0.6232886448882728469556013806140981614589691162109375;-0.7487619228159119177945513001759536564350128173828125;0.360102047606153996550659712738706730306148529052734375;0.86885043914286075317221502700704149901866912841796875;-0.56979940853644317488857495845877565443515777587890625;1.9584103859833053018491000329959206283092498779296875;-1.6617525670545336691219517888384871184825897216796875;-1.5744546945268182991384264823864214122295379638671875]
      mask Display: e = 0.06;c1 = [120 150 230]/255;c2 = ([120 150 230]+0)/383;c3 = ([120 150 230]+128)/383;patch([0 1 1 0],[0 0 1 1],c1);patch([0 1 1 1-e 1-e 0+e],[0 0 1 1-e 0+e 0+e],c2);patch([0 0 1 1-e 0+e 0+e],[0 1 1 1-e 1-e 0+e],c3);plot([0 1 1 0 0],[0 0 1 1 0]);disp('weights');
  "IW{2,1}(233,:)'" : Constant  Value=[0.0173525594985066596021017204520831000991165637969970703125;1.0481162261443854877285275506437756121158599853515625;0.319221749270883592419778551629860885441303253173828125;-0.2352881435526003317537657721914001740515232086181640625;-2.3441985971455867598933764384128153324127197265625;0.51575607399557477084073298101429827511310577392578125;-2.081753244663532509406422832398675382137298583984375;0.0289751306412936414369507787114343955181539058685302734375]
      mask Display: e = 0.06;c1 = [120 150 230]/255;c2 = ([120 150 230]+0)/383;c3 = ([120 150 230]+128)/383;patch([0 1 1 0],[0 0 1 1],c1);patch([0 1 1 1-e 1-e 0+e],[0 0 1 1-e 0+e 0+e],c2);patch([0 0 1 1-e 0+e 0+e],[0 1 1 1-e 1-e 0+e],c3);plot([0 1 1 0 0],[0 0 1 1 0]);disp('weights');
  "IW{2,1}(234,:)'" : Constant  Value=[-1.3159681249228005750495640313602052628993988037109375;1.0204199370387347922672915956354700028896331787109375;-0.56257995116517722777871313155628740787506103515625;-1.72858642034579634838564743404276669025421142578125;-1.9690558017797303858031909840065054595470428466796875;-0.36991225197593957663144692560308612883090972900390625;0.86872006361703746346591969995643012225627899169921875;0.03000904806360300824952247467081178911030292510986328125]
      mask Display: e = 0.06;c1 = [120 150 230]/255;c2 = ([120 150 230]+0)/383;c3 = ([120 150 230]+128)/383;patch([0 1 1 0],[0 0 1 1],c1);patch([0 1 1 1-e 1-e 0+e],[0 0 1 1-e 0+e 0+e],c2);patch([0 0 1 1-e 0+e 0+e],[0 1 1 1-e 1-e 0+e],c3);plot([0 1 1 0 0],[0 0 1 1 0]);disp('weights');
  "IW{2,1}(235,:)'" : Constant  Value=[1.36616760155419658673281446681357920169830322265625;1.3870065408612461954618311210651881992816925048828125;-0.225588467196818742710462402101256884634494781494140625;0.6064153941764647282042233200627379119396209716796875;1.7400337568408341670789241106831468641757965087890625;0.64908690805510638188735583753441460430622100830078125;-0.2166250899344415448144474112268653698265552520751953125;1.7252511330628215180382767357514239847660064697265625]
      mask Display: e = 0.06;c1 = [120 150 230]/255;c2 = ([120 150 230]+0)/383;c3 = ([120 150 230]+128)/383;patch([0 1 1 0],[0 0 1 1],c1);patch([0 1 1 1-e 1-e 0+e],[0 0 1 1-e 0+e 0+e],c2);patch([0 0 1 1-e 0+e 0+e],[0 1 1 1-e 1-e 0+e],c3);plot([0 1 1 0 0],[0 0 1 1 0]);disp('weights');
  "IW{2,1}(236,:)'" : Constant  Value=[-0.01273753889274030319522790222208641353063285350799560546875;-0.95025714314608744626156067170086316764354705810546875;-0.253481768548758645831497915423824451863765716552734375;1.6754690068428954585755263906321488320827484130859375;1.0460118381831211564758632448501884937286376953125;-1.065159442560359881468912135460413992404937744140625;-1.586436500476815947280329055502079427242279052734375;1.6084553043444047570886823450564406812191009521484375]
      mask Display: e = 0.06;c1 = [120 150 230]/255;c2 = ([120 150 230]+0)/383;c3 = ([120 150 230]+128)/383;patch([0 1 1 0],[0 0 1 1],c1);patch([0 1 1 1-e 1-e 0+e],[0 0 1 1-e 0+e 0+e],c2);patch([0 0 1 1-e 0+e 0+e],[0 1 1 1-e 1-e 0+e],c3);plot([0 1 1 0 0],[0 0 1 1 0]);disp('weights');
  "IW{2,1}(237,:)'" : Constant  Value=[-0.60606875348401667569220307996147312223911285400390625;-1.1689314668902006655315517491544596850872039794921875;-1.560754829858564729505587820312939584255218505859375;-1.1222910779043615558947522004018537700176239013671875;1.282862119051285443305232547572813928127288818359375;-0.33379779286001054483534744576900266110897064208984375;1.5145445900571292696668024291284382343292236328125;-1.2752100042335623442113501369021832942962646484375]
      mask Display: e = 0.06;c1 = [120 150 230]/255;c2 = ([120 150 230]+0)/383;c3 = ([120 150 230]+128)/383;patch([0 1 1 0],[0 0 1 1],c1);patch([0 1 1 1-e 1-e 0+e],[0 0 1 1-e 0+e 0+e],c2);patch([0 0 1 1-e 0+e 0+e],[0 1 1 1-e 1-e 0+e],c3);plot([0 1 1 0 0],[0 0 1 1 0]);disp('weights');
  "IW{2,1}(238,:)'" : Constant  Value=[1.5275787460153311680954857365577481687068939208984375;-0.67037288963324936919008223412674851715564727783203125;1.17507283829939712660461736959405243396759033203125;0.44896844104441113731951418230892159044742584228515625;-0.803801555763424602218947256915271282196044921875;1.2533262761146375385834517146577127277851104736328125;0.0958254501507147249395046628706040792167186737060546875;2.0955211458061029361488181166350841522216796875]
      mask Display: e = 0.06;c1 = [120 150 230]/255;c2 = ([120 150 230]+0)/383;c3 = ([120 150 230]+128)/383;patch([0 1 1 0],[0 0 1 1],c1);patch([0 1 1 1-e 1-e 0+e],[0 0 1 1-e 0+e 0+e],c2);patch([0 0 1 1-e 0+e 0+e],[0 1 1 1-e 1-e 0+e],c3);plot([0 1 1 0 0],[0 0 1 1 0]);disp('weights');
  "IW{2,1}(239,:)'" : Constant  Value=[-0.99480978147037524284002074637101031839847564697265625;1.511412659064708119416309273219667375087738037109375;1.9043551773848503838593160253367386758327484130859375;-0.2321330889564135746550022076917230151593685150146484375;1.18047348016894293465384180308319628238677978515625;-0.294196476998988709627980142613523639738559722900390625;1.2263712883754858129492504303925670683383941650390625;-1.0478239495485139887165360050857998430728912353515625]
      mask Display: e = 0.06;c1 = [120 150 230]/255;c2 = ([120 150 230]+0)/383;c3 = ([120 150 230]+128)/383;patch([0 1 1 0],[0 0 1 1],c1);patch([0 1 1 1-e 1-e 0+e],[0 0 1 1-e 0+e 0+e],c2);patch([0 0 1 1-e 0+e 0+e],[0 1 1 1-e 1-e 0+e],c3);plot([0 1 1 0 0],[0 0 1 1 0]);disp('weights');
  "IW{2,1}(24,:)'" : Constant  Value=[-1.3347236153250368051459417984005995094776153564453125;0.544055004395969543651290223351679742336273193359375;-0.581215819616144546699842976522631943225860595703125;-0.94988683883163671506366654284647665917873382568359375;-0.68351917886259039303098461459740065038204193115234375;1.1966914273801430024235514792962931096553802490234375;-1.8972470973184822895518664154224097728729248046875;1.444227363705493871748331002891063690185546875]
      mask Display: e = 0.06;c1 = [120 150 230]/255;c2 = ([120 150 230]+0)/383;c3 = ([120 150 230]+128)/383;patch([0 1 1 0],[0 0 1 1],c1);patch([0 1 1 1-e 1-e 0+e],[0 0 1 1-e 0+e 0+e],c2);patch([0 0 1 1-e 0+e 0+e],[0 1 1 1-e 1-e 0+e],c3);plot([0 1 1 0 0],[0 0 1 1 0]);disp('weights');
  "IW{2,1}(240,:)'" : Constant  Value=[-1.152563024838945349159757824963890016078948974609375;-0.520517020594430501745364381349645555019378662109375;-0.67472885989831132835803373382077552378177642822265625;-1.689962412270288982796273558051325380802154541015625;-1.126589127655068356403944562771357595920562744140625;1.7028891813288151713123852459830231964588165283203125;-0.54914976575974672190483261147164739668369293212890625;1.20570557546912393576121758087538182735443115234375]
      mask Display: e = 0.06;c1 = [120 150 230]/255;c2 = ([120 150 230]+0)/383;c3 = ([120 150 230]+128)/383;patch([0 1 1 0],[0 0 1 1],c1);patch([0 1 1 1-e 1-e 0+e],[0 0 1 1-e 0+e 0+e],c2);patch([0 0 1 1-e 0+e 0+e],[0 1 1 1-e 1-e 0+e],c3);plot([0 1 1 0 0],[0 0 1 1 0]);disp('weights');
  "IW{2,1}(241,:)'" : Constant  Value=[-1.4799941774846925302000499868881888687610626220703125;0.94866819426759196876020041599986143410205841064453125;-0.6028850129830980453249367201351560652256011962890625;1.356087566312369485643785083084367215633392333984375;-1.7129754563468513328672315765288658440113067626953125;1.5730565957264095455769847831106744706630706787109375;-0.0514844545558543753571711931726895272731781005859375;0.62198926406718613169033460508217103779315948486328125]
      mask Display: e = 0.06;c1 = [120 150 230]/255;c2 = ([120 150 230]+0)/383;c3 = ([120 150 230]+128)/383;patch([0 1 1 0],[0 0 1 1],c1);patch([0 1 1 1-e 1-e 0+e],[0 0 1 1-e 0+e 0+e],c2);patch([0 0 1 1-e 0+e 0+e],[0 1 1 1-e 1-e 0+e],c3);plot([0 1 1 0 0],[0 0 1 1 0]);disp('weights');
  "IW{2,1}(242,:)'" : Constant  Value=[-0.27071481113579209942798797783325426280498504638671875;1.4143816345271089662816166310221888124942779541015625;-1.1210627826836281339950573965325020253658294677734375;-1.3628101632623852434988975801388733088970184326171875;0.1403748692443008982966290432159439660608768463134765625;-1.4511690485563850661065998792764730751514434814453125;-1.5741400023290206267034818665706552565097808837890625;1.13563244839302068811548451776616275310516357421875]
      mask Display: e = 0.06;c1 = [120 150 230]/255;c2 = ([120 150 230]+0)/383;c3 = ([120 150 230]+128)/383;patch([0 1 1 0],[0 0 1 1],c1);patch([0 1 1 1-e 1-e 0+e],[0 0 1 1-e 0+e 0+e],c2);patch([0 0 1 1-e 0+e 0+e],[0 1 1 1-e 1-e 0+e],c3);plot([0 1 1 0 0],[0 0 1 1 0]);disp('weights');
  "IW{2,1}(243,:)'" : Constant  Value=[0.0854019787373082872594665104770683683454990386962890625;-0.1580118551228233136907164180229301564395427703857421875;1.6183189192549856105785011095576919615268707275390625;1.7536230184310122037771861869259737432003021240234375;0.379042678569220914397419619490392506122589111328125;1.571830760640730684229993130429647862911224365234375;-1.3171965114047454736834197319694794714450836181640625;0.96387676976835179321057012202800251543521881103515625]
      mask Display: e = 0.06;c1 = [120 150 230]/255;c2 = ([120 150 230]+0)/383;c3 = ([120 150 230]+128)/383;patch([0 1 1 0],[0 0 1 1],c1);patch([0 1 1 1-e 1-e 0+e],[0 0 1 1-e 0+e 0+e],c2);patch([0 0 1 1-e 0+e 0+e],[0 1 1 1-e 1-e 0+e],c3);plot([0 1 1 0 0],[0 0 1 1 0]);disp('weights');
  "IW{2,1}(244,:)'" : Constant  Value=[1.7889380979620781442207544387201778590679168701171875;-0.60500582621644960479301289524300955235958099365234375;0.3608227587454972962177635054104030132293701171875;-2.27164198646400006253998071770183742046356201171875;0.3844126447433051652069480041973292827606201171875;-0.37675268999086686250166167155839502811431884765625;0.53694356618311711581981171548250131309032440185546875;1.1453127369407827274017108720727264881134033203125]
      mask Display: e = 0.06;c1 = [120 150 230]/255;c2 = ([120 150 230]+0)/383;c3 = ([120 150 230]+128)/383;patch([0 1 1 0],[0 0 1 1],c1);patch([0 1 1 1-e 1-e 0+e],[0 0 1 1-e 0+e 0+e],c2);patch([0 0 1 1-e 0+e 0+e],[0 1 1 1-e 1-e 0+e],c3);plot([0 1 1 0 0],[0 0 1 1 0]);disp('weights');
  "IW{2,1}(245,:)'" : Constant  Value=[0.55584505674578965628285232014604844152927398681640625;0.6054282737431828653740240042679943144321441650390625;-1.9958542773360223865353191285976208746433258056640625;0.40853139040358588118806437705643475055694580078125;-1.03550353015714780013922791113145649433135986328125;-1.7364519252731993592675507898093201220035552978515625;-0.8956023479901535910840948417899198830127716064453125;1.1372945571537782516458037207485176622867584228515625]
      mask Display: e = 0.06;c1 = [120 150 230]/255;c2 = ([120 150 230]+0)/383;c3 = ([120 150 230]+128)/383;patch([0 1 1 0],[0 0 1 1],c1);patch([0 1 1 1-e 1-e 0+e],[0 0 1 1-e 0+e 0+e],c2);patch([0 0 1 1-e 0+e 0+e],[0 1 1 1-e 1-e 0+e],c3);plot([0 1 1 0 0],[0 0 1 1 0]);disp('weights');
  "IW{2,1}(246,:)'" : Constant  Value=[1.1303201738185160163396858479245565831661224365234375;1.15141970295984918948306585662066936492919921875;0.1006353677630207332782674711779691278934478759765625;2.454672572032486232984638263587839901447296142578125;-0.85286831085114467310148711476358585059642791748046875;0.97863833462851490541112298160442151129245758056640625;-0.061978479021380296354326588925687246955931186676025390625;0.94875106579904555648141695201047696173191070556640625]
      mask Display: e = 0.06;c1 = [120 150 230]/255;c2 = ([120 150 230]+0)/383;c3 = ([120 150 230]+128)/383;patch([0 1 1 0],[0 0 1 1],c1);patch([0 1 1 1-e 1-e 0+e],[0 0 1 1-e 0+e 0+e],c2);patch([0 0 1 1-e 0+e 0+e],[0 1 1 1-e 1-e 0+e],c3);plot([0 1 1 0 0],[0 0 1 1 0]);disp('weights');
  "IW{2,1}(247,:)'" : Constant  Value=[-0.96479873569583463055465699653723277151584625244140625;0.470512795847063680643174166107201017439365386962890625;1.28505727783237144734584944671951234340667724609375;-0.324069971757757258057353055846760980784893035888671875;1.1498343862880127108638816935126669704914093017578125;1.2977828406791698245825728008639998733997344970703125;1.5948340149156667866492398388800211250782012939453125;1.59928915194115806031049942248500883579254150390625]
      mask Display: e = 0.06;c1 = [120 150 230]/255;c2 = ([120 150 230]+0)/383;c3 = ([120 150 230]+128)/383;patch([0 1 1 0],[0 0 1 1],c1);patch([0 1 1 1-e 1-e 0+e],[0 0 1 1-e 0+e 0+e],c2);patch([0 0 1 1-e 0+e 0+e],[0 1 1 1-e 1-e 0+e],c3);plot([0 1 1 0 0],[0 0 1 1 0]);disp('weights');
  "IW{2,1}(248,:)'" : Constant  Value=[1.578910350332504375359121695510111749172210693359375;1.1190344861287557787221658145426772534847259521484375;1.445944370961894431815153438947163522243499755859375;-1.3140698628400786507341990727582015097141265869140625;1.467051389349393275551847182214260101318359375;-0.366836320697295992232511707697995007038116455078125;-0.2440367426959044461209913379207137040793895721435546875;-1.164052423469925212629050292889587581157684326171875]
      mask Display: e = 0.06;c1 = [120 150 230]/255;c2 = ([120 150 230]+0)/383;c3 = ([120 150 230]+128)/383;patch([0 1 1 0],[0 0 1 1],c1);patch([0 1 1 1-e 1-e 0+e],[0 0 1 1-e 0+e 0+e],c2);patch([0 0 1 1-e 0+e 0+e],[0 1 1 1-e 1-e 0+e],c3);plot([0 1 1 0 0],[0 0 1 1 0]);disp('weights');
  "IW{2,1}(249,:)'" : Constant  Value=[-1.875328856358359441713901105686090886592864990234375;-1.3876768948838529293965393662801943719387054443359375;1.0140971160439591347568466517259366810321807861328125;-1.6192941839407655191251933501916937530040740966796875;0.1488437464257293674219084778087562881410121917724609375;1.2450705431814672596857462849584408104419708251953125;-0.7966593686448655287080100606544874608516693115234375;-0.22435205033629956883345357709913514554500579833984375]
      mask Display: e = 0.06;c1 = [120 150 230]/255;c2 = ([120 150 230]+0)/383;c3 = ([120 150 230]+128)/383;patch([0 1 1 0],[0 0 1 1],c1);patch([0 1 1 1-e 1-e 0+e],[0 0 1 1-e 0+e 0+e],c2);patch([0 0 1 1-e 0+e 0+e],[0 1 1 1-e 1-e 0+e],c3);plot([0 1 1 0 0],[0 0 1 1 0]);disp('weights');
  "IW{2,1}(25,:)'" : Constant  Value=[-0.754085687695751349934880636283196508884429931640625;1.642181103341474379675446471082977950572967529296875;0.27529036638756176902376182624720968306064605712890625;1.98714437038190450124375274754129350185394287109375;0.7183173307726724576838250868604518473148345947265625;1.655640909036758312566917084041051566600799560546875;0.50721229532797218464423849582090042531490325927734375;-0.4670466967202420160987230701721273362636566162109375]
      mask Display: e = 0.06;c1 = [120 150 230]/255;c2 = ([120 150 230]+0)/383;c3 = ([120 150 230]+128)/383;patch([0 1 1 0],[0 0 1 1],c1);patch([0 1 1 1-e 1-e 0+e],[0 0 1 1-e 0+e 0+e],c2);patch([0 0 1 1-e 0+e 0+e],[0 1 1 1-e 1-e 0+e],c3);plot([0 1 1 0 0],[0 0 1 1 0]);disp('weights');
  "IW{2,1}(250,:)'" : Constant  Value=[-1.234980838725305840597457063267938792705535888671875;-1.6120922312676864152081179781816899776458740234375;0.0206656949263251225878956773840400273911654949188232421875;0.279763865542512923934026503047789447009563446044921875;-0.45041049653710896194525048485957086086273193359375;1.901811836170758329700447575305588543415069580078125;-1.7092527872137657229956175797269679605960845947265625;0.12126092759677910282167800914976396597921848297119140625]
      mask Display: e = 0.06;c1 = [120 150 230]/255;c2 = ([120 150 230]+0)/383;c3 = ([120 150 230]+128)/383;patch([0 1 1 0],[0 0 1 1],c1);patch([0 1 1 1-e 1-e 0+e],[0 0 1 1-e 0+e 0+e],c2);patch([0 0 1 1-e 0+e 0+e],[0 1 1 1-e 1-e 0+e],c3);plot([0 1 1 0 0],[0 0 1 1 0]);disp('weights');
  "IW{2,1}(251,:)'" : Constant  Value=[0.421008791349015865090876786780427210032939910888671875;-1.29652225373264773367054658592678606510162353515625;-0.8832342861338682293848023618920706212520599365234375;1.412020838201837324987764077377505600452423095703125;1.57350086911555475666091297171078622341156005859375;-1.2094230285506475386370084379450418055057525634765625;0.9884190847860174766736918172682635486125946044921875;-1.197083928948013298310115715139545500278472900390625]
      mask Display: e = 0.06;c1 = [120 150 230]/255;c2 = ([120 150 230]+0)/383;c3 = ([120 150 230]+128)/383;patch([0 1 1 0],[0 0 1 1],c1);patch([0 1 1 1-e 1-e 0+e],[0 0 1 1-e 0+e 0+e],c2);patch([0 0 1 1-e 0+e 0+e],[0 1 1 1-e 1-e 0+e],c3);plot([0 1 1 0 0],[0 0 1 1 0]);disp('weights');
  "IW{2,1}(252,:)'" : Constant  Value=[-1.9426439968464936924874564283527433872222900390625;1.640454988807554581597969445283524692058563232421875;-0.72665200390230466620522520315716974437236785888671875;-1.526160283943448714438773095025680959224700927734375;-0.470933578064877955693390276792342774569988250732421875;-0.58298202970808266076829795565572567284107208251953125;0.46843915869012497932288852098281495273113250732421875;-0.9285679644148425726513096378766931593418121337890625]
      mask Display: e = 0.06;c1 = [120 150 230]/255;c2 = ([120 150 230]+0)/383;c3 = ([120 150 230]+128)/383;patch([0 1 1 0],[0 0 1 1],c1);patch([0 1 1 1-e 1-e 0+e],[0 0 1 1-e 0+e 0+e],c2);patch([0 0 1 1-e 0+e 0+e],[0 1 1 1-e 1-e 0+e],c3);plot([0 1 1 0 0],[0 0 1 1 0]);disp('weights');
  "IW{2,1}(253,:)'" : Constant  Value=[0.8857454921067120512390147268888540565967559814453125;1.0524354215880167284780100089847110211849212646484375;0.11651735783166107529584820667878375388681888580322265625;0.53565919751482471422576736586051993072032928466796875;1.53983513954512307719824093510396778583526611328125;-1.3176282567187482808179765925160609185695648193359375;1.501252201783066286822077017859555780887603759765625;1.501643213924673592174485747818835079669952392578125]
      mask Display: e = 0.06;c1 = [120 150 230]/255;c2 = ([120 150 230]+0)/383;c3 = ([120 150 230]+128)/383;patch([0 1 1 0],[0 0 1 1],c1);patch([0 1 1 1-e 1-e 0+e],[0 0 1 1-e 0+e 0+e],c2);patch([0 0 1 1-e 0+e 0+e],[0 1 1 1-e 1-e 0+e],c3);plot([0 1 1 0 0],[0 0 1 1 0]);disp('weights');
  "IW{2,1}(254,:)'" : Constant  Value=[-0.53392224642707974968658390935161150991916656494140625;-1.4929130064335078831305736457579769194126129150390625;-2.038694389684057028944152989424765110015869140625;-0.55376020045128060420580595746287144720554351806640625;-0.26254624388593506001399191518430598080158233642578125;-1.24406749999441412768419468193314969539642333984375;0.1161767152671029090793552995819482021033763885498046875;1.5229961469595725276349185151048004627227783203125]
      mask Display: e = 0.06;c1 = [120 150 230]/255;c2 = ([120 150 230]+0)/383;c3 = ([120 150 230]+128)/383;patch([0 1 1 0],[0 0 1 1],c1);patch([0 1 1 1-e 1-e 0+e],[0 0 1 1-e 0+e 0+e],c2);patch([0 0 1 1-e 0+e 0+e],[0 1 1 1-e 1-e 0+e],c3);plot([0 1 1 0 0],[0 0 1 1 0]);disp('weights');
  "IW{2,1}(255,:)'" : Constant  Value=[-1.7464560114748095553949269742588512599468231201171875;0.8933561626841057812242752333986572921276092529296875;0.298530452919288313839984994046972133219242095947265625;-1.0243289986431698412872037806664593517780303955078125;-1.091714310140373012103509609005413949489593505859375;2.07835353578775627880759202525950968265533447265625;-0.89155802693860286556315486450330354273319244384765625;-0.342035025848102469669953507036552764475345611572265625]
      mask Display: e = 0.06;c1 = [120 150 230]/255;c2 = ([120 150 230]+0)/383;c3 = ([120 150 230]+128)/383;patch([0 1 1 0],[0 0 1 1],c1);patch([0 1 1 1-e 1-e 0+e],[0 0 1 1-e 0+e 0+e],c2);patch([0 0 1 1-e 0+e 0+e],[0 1 1 1-e 1-e 0+e],c3);plot([0 1 1 0 0],[0 0 1 1 0]);disp('weights');
  "IW{2,1}(256,:)'" : Constant  Value=[-0.152501495180584478728036401662393473088741302490234375;-1.844754216614143071950593366636894643306732177734375;-0.14150604882608430745705163644743151962757110595703125;-1.683414782432349543483951492817141115665435791015625;-1.8940580950042027463808835818781517446041107177734375;1.0264708919394076591657949393265880644321441650390625;-0.3150687096569837475357189759961329400539398193359375;-0.268719412502356702621142403586418367922306060791015625]
      mask Display: e = 0.06;c1 = [120 150 230]/255;c2 = ([120 150 230]+0)/383;c3 = ([120 150 230]+128)/383;patch([0 1 1 0],[0 0 1 1],c1);patch([0 1 1 1-e 1-e 0+e],[0 0 1 1-e 0+e 0+e],c2);patch([0 0 1 1-e 0+e 0+e],[0 1 1 1-e 1-e 0+e],c3);plot([0 1 1 0 0],[0 0 1 1 0]);disp('weights');
  "IW{2,1}(257,:)'" : Constant  Value=[1.318412508728698639970389194786548614501953125;-1.6926035292757557471077234367839992046356201171875;1.637140106075978263078241070616059005260467529296875;-1.1485786974768876778085768819437362253665924072265625;-0.290123280731632793294494376823422499001026153564453125;-0.82572175305491890551223832517280243337154388427734375;-0.73072407744742984281316466876887716352939605712890625;1.0671845113473594768294105961103923618793487548828125]
      mask Display: e = 0.06;c1 = [120 150 230]/255;c2 = ([120 150 230]+0)/383;c3 = ([120 150 230]+128)/383;patch([0 1 1 0],[0 0 1 1],c1);patch([0 1 1 1-e 1-e 0+e],[0 0 1 1-e 0+e 0+e],c2);patch([0 0 1 1-e 0+e 0+e],[0 1 1 1-e 1-e 0+e],c3);plot([0 1 1 0 0],[0 0 1 1 0]);disp('weights');
  "IW{2,1}(258,:)'" : Constant  Value=[-1.890575690785672779981041458086110651493072509765625;-0.047546284495999978358948823142782202921807765960693359375;-1.5702137813283416623022503699758090078830718994140625;-0.26048623173423790522207355024875141680240631103515625;0.5562906300168541928741205992992036044597625732421875;0.11772910008703858786294205174272065050899982452392578125;-1.9749745807068912473170030352775938808917999267578125;-0.887767982004268763063237202004529535770416259765625]
      mask Display: e = 0.06;c1 = [120 150 230]/255;c2 = ([120 150 230]+0)/383;c3 = ([120 150 230]+128)/383;patch([0 1 1 0],[0 0 1 1],c1);patch([0 1 1 1-e 1-e 0+e],[0 0 1 1-e 0+e 0+e],c2);patch([0 0 1 1-e 0+e 0+e],[0 1 1 1-e 1-e 0+e],c3);plot([0 1 1 0 0],[0 0 1 1 0]);disp('weights');
  "IW{2,1}(259,:)'" : Constant  Value=[0.27799020619940417731186244054697453975677490234375;-0.599296521262968173715535158407874405384063720703125;2.22029859257213768586325386422686278820037841796875;0.71966442582228229429830435037729330360889434814453125;1.5153777633471487984451187003287486732006072998046875;-0.77625479019154308701899935840629041194915771484375;0.69782502371072097080428875415236689150333404541015625;1.3976941426588478378789659473113715648651123046875]
      mask Display: e = 0.06;c1 = [120 150 230]/255;c2 = ([120 150 230]+0)/383;c3 = ([120 150 230]+128)/383;patch([0 1 1 0],[0 0 1 1],c1);patch([0 1 1 1-e 1-e 0+e],[0 0 1 1-e 0+e 0+e],c2);patch([0 0 1 1-e 0+e 0+e],[0 1 1 1-e 1-e 0+e],c3);plot([0 1 1 0 0],[0 0 1 1 0]);disp('weights');
  "IW{2,1}(26,:)'" : Constant  Value=[0.7107823001892865644180119488737545907497406005859375;1.1817744151516358375175741457496769726276397705078125;-1.3924335901025057804503148872754536569118499755859375;-0.132285482567261747366416102522634901106357574462890625;-1.4049992182996984269038875936530530452728271484375;1.17367306336583876458234954043291509151458740234375;1.2752596054543074988174566897214390337467193603515625;1.5089586252231743657148399506695568561553955078125]
      mask Display: e = 0.06;c1 = [120 150 230]/255;c2 = ([120 150 230]+0)/383;c3 = ([120 150 230]+128)/383;patch([0 1 1 0],[0 0 1 1],c1);patch([0 1 1 1-e 1-e 0+e],[0 0 1 1-e 0+e 0+e],c2);patch([0 0 1 1-e 0+e 0+e],[0 1 1 1-e 1-e 0+e],c3);plot([0 1 1 0 0],[0 0 1 1 0]);disp('weights');
  "IW{2,1}(260,:)'" : Constant  Value=[-1.0813447018700179658168281093821860849857330322265625;-0.7917954674598763897819253543275408446788787841796875;-0.9933771895396568130109926642035134136676788330078125;1.972046303939056333121015995857305824756622314453125;0.0132475677344050003780839830369586707092821598052978515625;-1.3784757399091909224608798467670567333698272705078125;1.27859358563055192092861034325323998928070068359375;-0.74394630823288265819570597159327007830142974853515625]
      mask Display: e = 0.06;c1 = [120 150 230]/255;c2 = ([120 150 230]+0)/383;c3 = ([120 150 230]+128)/383;patch([0 1 1 0],[0 0 1 1],c1);patch([0 1 1 1-e 1-e 0+e],[0 0 1 1-e 0+e 0+e],c2);patch([0 0 1 1-e 0+e 0+e],[0 1 1 1-e 1-e 0+e],c3);plot([0 1 1 0 0],[0 0 1 1 0]);disp('weights');
